simulink model "active_vehicle_ESP_Control"  (R2020a)
settings: Solver=ode4  StartTime=0.0  StopTime=inf  FixedStep=1e-3  RelTol=1e-3
InitFcn:
  | clear mex
model workspace (MAT data in the model file):
  inChnlList : object (value not decoded)
  inChnlListInternal : object (value not decoded)
  outChnlList : object (value not decoded)
  outChnlListInternal : object (value not decoded)
undefined symbols (not defined in the file or in its folder): DiscIntNeverNeededParam, vicrt_initcallback, vicrt_initmexcallback, vicrt_inputfile, vicrt_simulationmanager
libraries: simulink x1
(part 4 of 6)

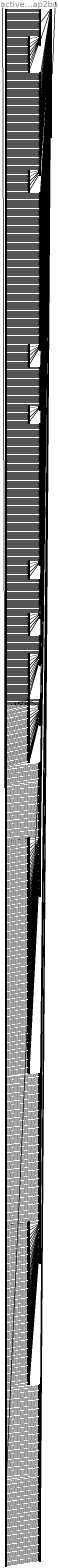
== system active_vehicle_ESP_Control/Vehicle/VI-CarRealTime/Output_Bus/IOmap2bus ==
  In : Inport
  ABS_Activity : BusCreator  Inputs=4
  Actual_Tread_Speed : BusCreator  Inputs=4
  Aggregate_Force_At_Wheel : BusCreator  Inputs=4
  Alpha : BusCreator  Inputs=4
  Animator_Widget : BusCreator  Inputs=2
  Auxiliary_Roll_Force : BusCreator  Inputs=4
  Auxiliary_Roll_Force_at_element : BusCreator  Inputs=2
  Auxiliary_Roll_deformation_at_element : BusCreator  Inputs=2
  Brake : BusCreator  Inputs=8
  Brake_Moment : BusCreator  Inputs=4
  Caster_Angle : BusCreator  Inputs=2
  Chamber_Pressure : BusCreator  Inputs=4
  Contact_Flag : BusCreator  Inputs=4
  Contact_Patch_Global_X : BusCreator  Inputs=4
  Contact_Patch_Global_X1 : BusCreator  Inputs=4
  Contact_Patch_Global_Y : BusCreator  Inputs=4
  Contact_Patch_Global_Y1 : BusCreator  Inputs=4
  Contact_Patch_Global_Z : BusCreator  Inputs=4
  Contact_Patch_Global_Z1 : BusCreator  Inputs=4
  Contact_Patch_Normal_X : BusCreator  Inputs=4
  Contact_Patch_Normal_Y : BusCreator  Inputs=4
  Contact_Patch_Normal_Z : BusCreator  Inputs=4
  Damper : BusCreator  Inputs=5
  Demux : Demux  Outputs=1374
  Drive_Moment : BusCreator  Inputs=4
  Effective_Closing_Speed : BusCreator  Inputs=4
  Effective_Penetration : BusCreator  Inputs=4
  Effective_Rolling_Radius : BusCreator  Inputs=4
  Equivalent_Tread_Speed : BusCreator  Inputs=4
  Euler_Roll : BusCreator  Inputs=4
  External_Friction_Scale_Factor : BusCreator  Inputs=4
  Force_At_Bumper : BusCreator  Inputs=4
  Force_At_Bumper1 : BusCreator  Inputs=4
  Force_At_Damper : BusCreator  Inputs=4
  Force_At_Inerter : BusCreator  Inputs=4
  Force_At_Spring : BusCreator  Inputs=4
  Force_At_Wheel{,1..4} (5 alike) : BusCreator  Inputs=4
  Force_Aux_At_Wheel : BusCreator  Inputs=4
  Global_Omega_X : BusCreator  Inputs=4
  Global_Omega_Y : BusCreator  Inputs=4
  Global_Omega_Z : BusCreator  Inputs=4
  Global_Vx : BusCreator  Inputs=4
  Global_Vy : BusCreator  Inputs=4
  Global_Vz : BusCreator  Inputs=4
  Global_X : BusCreator  Inputs=4
  Global_Y : BusCreator  Inputs=4
  Global_Z : BusCreator  Inputs=4
  Ground_Surface_Contact_Patch_Vx : BusCreator  Inputs=4
  Ground_Surface_Contact_Patch_Vy : BusCreator  Inputs=4
  Ground_Surface_Force_X : BusCreator  Inputs=4
  Ground_Surface_Force_Y : BusCreator  Inputs=4
  Ground_Surface_Force_Z : BusCreator  Inputs=4
  Ground_Surface_Gyroscopic_Moment : BusCreator  Inputs=4
  Ground_Surface_Kappa_Fy : BusCreator  Inputs=4
  Ground_Surface_Moment_X : BusCreator  Inputs=4
  Ground_Surface_Moment_Y : BusCreator  Inputs=4
  Ground_Surface_Moment_Z : BusCreator  Inputs=4
  Ground_Surface_Peak_Friction_X : BusCreator  Inputs=4
  Ground_Surface_Peak_Friction_Y : BusCreator  Inputs=4
  Ground_Surface_Residual_Torque : BusCreator  Inputs=4
  Ground_Surface_Wheel_Center_Vx : BusCreator  Inputs=4
  Gyro : BusCreator  Inputs=10
  Hook_rear : BusCreator  Inputs=18
  Hub_Carrier_Force_Global_X : BusCreator  Inputs=4
  Hub_Carrier_Force_Global_Y : BusCreator  Inputs=4
  Hub_Carrier_Force_Global_Z : BusCreator  Inputs=4
  Hub_Carrier_Force_Local_X : BusCreator  Inputs=4
  Hub_Carrier_Force_Local_Y : BusCreator  Inputs=4
  Hub_Carrier_Force_Local_Z : BusCreator  Inputs=4
  Hub_Carrier_Moment_Global_X : BusCreator  Inputs=4
  Hub_Carrier_Moment_Global_Y : BusCreator  Inputs=4
  Hub_Carrier_Moment_Global_Z : BusCreator  Inputs=4
  Hub_Carrier_Moment_Local_X : BusCreator  Inputs=4
  Hub_Carrier_Moment_Local_Y : BusCreator  Inputs=4
  Hub_Carrier_Moment_Local_Z : BusCreator  Inputs=4
  Hub_Carrier_Omega_X : BusCreator  Inputs=4
  Hub_Carrier_Omega_Y : BusCreator  Inputs=4
  Hub_Carrier_Omega_Z : BusCreator  Inputs=4
  Hub_Carrier_Vx : BusCreator  Inputs=4
  Hub_Carrier_Vy : BusCreator  Inputs=4
  Hub_Carrier_Vz : BusCreator  Inputs=4
  Inclination : BusCreator  Inputs=4
  Inerter : BusCreator  Inputs=5
  Inst_Stiff_Deflection : BusCreator  Inputs=4
  Inst_Stiff_Force : BusCreator  Inputs=4
  Jounce{,1..5} (6 alike) : BusCreator  Inputs=4
  Jounce_Acceleration{,1..3} (4 alike) : BusCreator  Inputs=4
  Jounce_Bumper : BusCreator  Inputs=4
  Jounce_Rate{,1..5} (6 alike) : BusCreator  Inputs=4
  Kingpin_Moment : BusCreator  Inputs=1
  Kingpin_Moment1 : BusCreator  Inputs=2
  Lateral_Relaxation_Length : BusCreator  Inputs=4
  Lateral_Slip_With_Lag : BusCreator  Inputs=4
  Lateral_Slip_Without_Lag : BusCreator  Inputs=4
  Loaded_Radius : BusCreator  Inputs=4
  Locked_Damper_Moment : BusCreator  Inputs=4
  Locked_Moment : BusCreator  Inputs=4
  Locked_Spring_Moment : BusCreator  Inputs=4
  Locked_Switch : BusCreator  Inputs=4
  Lockup_Rotation : BusCreator  Inputs=4
  Longitudinal_Relaxation_Length : BusCreator  Inputs=4
  Longitudinal_Slip_With_Lag : BusCreator  Inputs=4
  Longitudinal_Slip_Without_Lag : BusCreator  Inputs=4
  Moment_Arm_Of_Fx : BusCreator  Inputs=4
  Off_Road_Flag : BusCreator  Inputs=4
  Omega : BusCreator  Inputs=4
  OutputBus : BusCreator  Inputs=113
  PID_CW_At_Spring : BusCreator  Inputs=4
  PID_PH_At_Spring : BusCreator  Inputs=4
  PID_RH_At_Spring : BusCreator  Inputs=4
  Phi : BusCreator  Inputs=4
  Pitch : BusCreator  Inputs=4
  Pneumatic_Trail : BusCreator  Inputs=4
  Pressure : BusCreator  Inputs=4
  Psi : BusCreator  Inputs=4
  Rebound_Bumper : BusCreator  Inputs=4
  Road : BusCreator  Inputs=5
  Road_Material : BusCreator  Inputs=4
  Road_friction : BusCreator  Inputs=4
  Roll : BusCreator  Inputs=2
  Roll_Center_Height : BusCreator  Inputs=2
  Roll_Center_Lateral_Displacement : BusCreator  Inputs=2
  Rotation : BusCreator  Inputs=4
  Sensor : BusCreator  Inputs=16
  Side_View_Angle : BusCreator  Inputs=4
  Spindle_Steer : BusCreator  Inputs=4
  Spring : BusCreator  Inputs=10
  Steering_Instant_Axis_Rotation : BusCreator  Inputs=2
  Steering_System : BusCreator  Inputs=7
  Suspension : BusCreator  Inputs=16
  System : BusCreator  Inputs=17
  System_Mass_Center : BusCreator  Inputs=13
  Temperature_1 : BusCreator  Inputs=4
  Temperature_2 : BusCreator  Inputs=4
  Temperature_3 : BusCreator  Inputs=4
  Theta : BusCreator  Inputs=4
  TieRod_Force_Left : BusCreator  Inputs=3
  TieRod_Force_Right : BusCreator  Inputs=3
  Tire : BusCreator  Inputs=52
  User_Input_Contact_Patch_Global_Z_Perturbation : BusCreator  Inputs=4
  Vehicle : BusCreator  Inputs=46
  Vehicle_States : BusCreator  Inputs=20
  Wheel : BusCreator  Inputs=37
  Yaw : BusCreator  Inputs=4
  aero_forces : BusCreator  Inputs=24
  base_acceleration : BusCreator  Inputs=4
  base_deformation : BusCreator  Inputs=4
  base_velocity : BusCreator  Inputs=4
  bul_jounce_stop_data : BusCreator  Inputs=6
  bul_rebound_stop_data : BusCreator  Inputs=6
  bur_jounce_stop_data : BusCreator  Inputs=6
  bur_rebound_stop_data : BusCreator  Inputs=6
  bus_dmp_jounce_stop_data : BusCreator  Inputs=6
  bus_ins_jounce_stop_data : BusCreator  Inputs=6
  bus_roll_dmp_jounce_stop_data : BusCreator  Inputs=6
  bus_spr_jounce_stop_data : BusCreator  Inputs=6
  chassis_accelerations : BusCreator  Inputs=6
  chassis_displacements : BusCreator  Inputs=9
  chassis_velocities : BusCreator  Inputs=6
  clutch : BusCreator  Inputs=8
  condition_sensors : BusCreator  Inputs=1
  cp_force_lateralFL : BusCreator  Inputs=3
  cp_force_lateralFR : BusCreator  Inputs=3
  cp_force_lateralRL : BusCreator  Inputs=3
  cp_force_lateralRR : BusCreator  Inputs=3
  cp_force_longitudinalFL : BusCreator  Inputs=3
  cp_force_longitudinalFR : BusCreator  Inputs=3
  cp_force_longitudinalRL : BusCreator  Inputs=3
  cp_force_longitudinalRR : BusCreator  Inputs=3
  cp_force_normalFL : BusCreator  Inputs=3
  cp_force_normalFR : BusCreator  Inputs=3
  cp_force_normalRL : BusCreator  Inputs=3
  cp_force_normalRR : BusCreator  Inputs=3
  cross_weight : BusCreator  Inputs=4
  dal_ride_damper_data : BusCreator  Inputs=4
  dar_ride_damper_data : BusCreator  Inputs=4
  das_ride_damper_data : BusCreator  Inputs=6
  das_roll_damper_data : BusCreator  Inputs=8
  das_third_damper_data : BusCreator  Inputs=6
  differential_central : BusCreator  Inputs=7
  differential_front : BusCreator  Inputs=7
  differential_rear : BusCreator  Inputs=7
  differential_speeds : BusCreator  Inputs=9
  differential_torques : BusCreator  Inputs=9
  driver_demands : BusCreator  Inputs=7
  driving_machine_monitor : BusCreator  Inputs=15
  engine : BusCreator  Inputs=11
  fuel_consumption : BusCreator  Inputs=4
  ges_chassis_XFORM : BusCreator  Inputs=6
  ges_hub_XFORMFL : BusCreator  Inputs=6
  ges_hub_XFORMFR : BusCreator  Inputs=6
  ges_hub_XFORMRL : BusCreator  Inputs=6
  ges_hub_XFORMRR : BusCreator  Inputs=6
  hub2cp_XFORMFL : BusCreator  Inputs=3
  hub2cp_XFORMFR : BusCreator  Inputs=3
  hub2cp_XFORMRL : BusCreator  Inputs=3
  hub2cp_XFORMRR : BusCreator  Inputs=3
  hub_center_accx : BusCreator  Inputs=4
  hub_center_accy : BusCreator  Inputs=4
  hub_center_accz : BusCreator  Inputs=4
  inl_ride_inerter_data : BusCreator  Inputs=6
  inr_ride_inerter_data : BusCreator  Inputs=6
  ins_inerter_data : BusCreator  Inputs=10
  jfs_torsional_stiffness_data : BusCreator  Inputs=12
  motor_to_central_differential : BusCreator  Inputs=11
  motor_to_clutch : BusCreator  Inputs=11
  motor_to_front_differential : BusCreator  Inputs=11
  motor_to_front_left_wheel : BusCreator  Inputs=11
  motor_to_front_right_wheel : BusCreator  Inputs=11
  motor_to_gearbox : BusCreator  Inputs=11
  motor_to_rear_differential : BusCreator  Inputs=11
  motor_to_rear_left_wheel : BusCreator  Inputs=11
  motor_to_rear_right_wheel : BusCreator  Inputs=11
  nsl_ride_spring_data : BusCreator  Inputs=6
  nsr_ride_spring_data : BusCreator  Inputs=6
  nss_ride_spring_data : BusCreator  Inputs=10
  res_dmp_rebound_stop_data : BusCreator  Inputs=6
  res_ins_rebound_stop_data : BusCreator  Inputs=6
  res_roll_dmp_rebound_stop_data : BusCreator  Inputs=6
  res_spr_rebound_stop_data : BusCreator  Inputs=6
  rhl_front_setup_sensor_data : BusCreator  Inputs=1
  rhl_rear_setup_sensor_data : BusCreator  Inputs=1
  rhr_front_setup_sensor_data : BusCreator  Inputs=1
  rhr_rear_setup_sensor_data : BusCreator  Inputs=1
  rhs_front_setup_sensor_data : BusCreator  Inputs=1
  rhs_rear_setup_sensor_data : BusCreator  Inputs=1
  til_wheel_tire_forces : BusCreator  Inputs=18
  til_wheel_tire_kinematics : BusCreator  Inputs=9
  til_wheel_tire_rolling_states : BusCreator  Inputs=9
  tir_wheel_tire_forces : BusCreator  Inputs=18
  tir_wheel_tire_kinematics : BusCreator  Inputs=9
  tir_wheel_tire_rolling_states : BusCreator  Inputs=9
  torque_converter : BusCreator  Inputs=9
  transmission : BusCreator  Inputs=10
  ues_third_spring_data : BusCreator  Inputs=6
  upright_accelerometer : BusCreator  Inputs=4
  wheel_angles : BusCreator  Inputs=24
  wheel_center_dispx : BusCreator  Inputs=4
  wheel_center_dispy : BusCreator  Inputs=4
  wheel_center_dispz : BusCreator  Inputs=4
  whl_front_wheel_XFORM : BusCreator  Inputs=9
  whl_rear_wheel_XFORM : BusCreator  Inputs=9
  whl_twin_rear_wheel_XFORM : BusCreator  Inputs=9
  whr_front_wheel_XFORM : BusCreator  Inputs=9
  whr_rear_wheel_XFORM : BusCreator  Inputs=9
  whr_twin_rear_wheel_XFORM : BusCreator  Inputs=9
  Out : Outport
  wires:
  In/1 -> Demux/1
  OutputBus/1 -> Out/1  "OutputBus"
  aero_forces/1 -> OutputBus/1  "aero_forces"
  Demux/1 -> aero_forces/1  "aero_balance"
  Demux/2 -> aero_forces/2  "center_downforce"
  Demux/3 -> aero_forces/3  "center_sideforce"
  Demux/4 -> aero_forces/4  "drag_arm"
  Demux/5 -> aero_forces/5  "drag_force"
  Demux/6 -> aero_forces/6  "drag_force_front"
  Demux/7 -> aero_forces/7  "drag_force_rear"
  Demux/8 -> aero_forces/8  "drag_torque"
  Demux/9 -> aero_forces/9  "front_downforce"
  Demux/10 -> aero_forces/10  "front_sideforce"
  Demux/11 -> aero_forces/11  "height_auxiliary"
  Demux/12 -> aero_forces/12  "height_front"
  Demux/13 -> aero_forces/13  "height_rear"
  Demux/14 -> aero_forces/14  "lateral_velocity"
  Demux/15 -> aero_forces/15  "longitudinal_velocity"
  Demux/16 -> aero_forces/16  "pitch"
  Demux/17 -> aero_forces/17  "rear_downforce"
  Demux/18 -> aero_forces/18  "rear_sideforce"
  Demux/19 -> aero_forces/19  "roll"
  Demux/20 -> aero_forces/20  "roll_torque"
  Demux/21 -> aero_forces/21  "side_slip"
  Demux/22 -> aero_forces/22  "steer"
  Demux/23 -> aero_forces/23  "vertical_velocity"
  Demux/24 -> aero_forces/24  "yaw_torque"
  Brake/1 -> OutputBus/2  "Brake"
  ABS_Activity/1 -> Brake/1  "ABS_Activity"
  Demux/25 -> ABS_Activity/1  "L1"
  Demux/26 -> ABS_Activity/2  "L2"
  Demux/27 -> ABS_Activity/3  "R1"
  Demux/28 -> ABS_Activity/4  "R2"
  Brake_Moment/1 -> Brake/2  "Brake_Moment"
  Demux/29 -> Brake_Moment/1  "L1"
  Demux/30 -> Brake_Moment/2  "L2"
  Demux/31 -> Brake_Moment/3  "R1"
  Demux/32 -> Brake_Moment/4  "R2"
  Chamber_Pressure/1 -> Brake/3  "Chamber_Pressure"
  Demux/33 -> Chamber_Pressure/1  "L1"
  Demux/34 -> Chamber_Pressure/2  "L2"
  Demux/35 -> Chamber_Pressure/3  "R1"
  Demux/36 -> Chamber_Pressure/4  "R2"
  Locked_Damper_Moment/1 -> Brake/4  "Locked_Damper_Moment"
  Demux/37 -> Locked_Damper_Moment/1  "L1"
  Demux/38 -> Locked_Damper_Moment/2  "L2"
  Demux/39 -> Locked_Damper_Moment/3  "R1"
  Demux/40 -> Locked_Damper_Moment/4  "R2"
  Locked_Moment/1 -> Brake/5  "Locked_Moment"
  Demux/41 -> Locked_Moment/1  "L1"
  Demux/42 -> Locked_Moment/2  "L2"
  Demux/43 -> Locked_Moment/3  "R1"
  Demux/44 -> Locked_Moment/4  "R2"
  Locked_Spring_Moment/1 -> Brake/6  "Locked_Spring_Moment"
  Demux/45 -> Locked_Spring_Moment/1  "L1"
  Demux/46 -> Locked_Spring_Moment/2  "L2"
  Demux/47 -> Locked_Spring_Moment/3  "R1"
  Demux/48 -> Locked_Spring_Moment/4  "R2"
  Locked_Switch/1 -> Brake/7  "Locked_Switch"
  Demux/49 -> Locked_Switch/1  "L1"
  Demux/50 -> Locked_Switch/2  "L2"
  Demux/51 -> Locked_Switch/3  "R1"
  Demux/52 -> Locked_Switch/4  "R2"
  Lockup_Rotation/1 -> Brake/8  "Lockup_Rotation"
  Demux/53 -> Lockup_Rotation/1  "L1"
  Demux/54 -> Lockup_Rotation/2  "L2"
  Demux/55 -> Lockup_Rotation/3  "R1"
  Demux/56 -> Lockup_Rotation/4  "R2"
  bul_jounce_stop_data/1 -> OutputBus/3  "bul_jounce_stop_data"
  Demux/57 -> bul_jounce_stop_data/1  "force_front"
  Demux/58 -> bul_jounce_stop_data/2  "force_rear"
  Demux/59 -> bul_jounce_stop_data/3  "jounce_front"
  Demux/60 -> bul_jounce_stop_data/4  "jounce_rear"
  Demux/61 -> bul_jounce_stop_data/5  "velocity_front"
  Demux/62 -> bul_jounce_stop_data/6  "velocity_rear"
  bul_rebound_stop_data/1 -> OutputBus/4  "bul_rebound_stop_data"
  Demux/63 -> bul_rebound_stop_data/1  "force_front"
  Demux/64 -> bul_rebound_stop_data/2  "force_rear"
  Demux/65 -> bul_rebound_stop_data/3  "jounce_front"
  Demux/66 -> bul_rebound_stop_data/4  "jounce_rear"
  Demux/67 -> bul_rebound_stop_data/5  "velocity_front"
  Demux/68 -> bul_rebound_stop_data/6  "velocity_rear"
  bur_jounce_stop_data/1 -> OutputBus/5  "bur_jounce_stop_data"
  Demux/69 -> bur_jounce_stop_data/1  "force_front"
  Demux/70 -> bur_jounce_stop_data/2  "force_rear"
  Demux/71 -> bur_jounce_stop_data/3  "jounce_front"
  Demux/72 -> bur_jounce_stop_data/4  "jounce_rear"
  Demux/73 -> bur_jounce_stop_data/5  "velocity_front"
  Demux/74 -> bur_jounce_stop_data/6  "velocity_rear"
  bur_rebound_stop_data/1 -> OutputBus/6  "bur_rebound_stop_data"
  Demux/75 -> bur_rebound_stop_data/1  "force_front"
  Demux/76 -> bur_rebound_stop_data/2  "force_rear"
  Demux/77 -> bur_rebound_stop_data/3  "jounce_front"
  Demux/78 -> bur_rebound_stop_data/4  "jounce_rear"
  Demux/79 -> bur_rebound_stop_data/5  "velocity_front"
  Demux/80 -> bur_rebound_stop_data/6  "velocity_rear"
  bus_dmp_jounce_stop_data/1 -> OutputBus/7  "bus_dmp_jounce_stop_data"
  Demux/81 -> bus_dmp_jounce_stop_data/1  "displacement_front"
  Demux/82 -> bus_dmp_jounce_stop_data/2  "displacement_rear"
  Demux/83 -> bus_dmp_jounce_stop_data/3  "force_front"
  Demux/84 -> bus_dmp_jounce_stop_data/4  "force_rear"
  Demux/85 -> bus_dmp_jounce_stop_data/5  "velocity_front"
  Demux/86 -> bus_dmp_jounce_stop_data/6  "velocity_rear"
  bus_ins_jounce_stop_data/1 -> OutputBus/8  "bus_ins_jounce_stop_data"
  Demux/87 -> bus_ins_jounce_stop_data/1  "displacement_front"
  Demux/88 -> bus_ins_jounce_stop_data/2  "displacement_rear"
  Demux/89 -> bus_ins_jounce_stop_data/3  "force_front"
  Demux/90 -> bus_ins_jounce_stop_data/4  "force_rear"
  Demux/91 -> bus_ins_jounce_stop_data/5  "velocity_front"
  Demux/92 -> bus_ins_jounce_stop_data/6  "velocity_rear"
  bus_roll_dmp_jounce_stop_data/1 -> OutputBus/9  "bus_roll_dmp_jounce_stop_data"
  Demux/93 -> bus_roll_dmp_jounce_stop_data/1  "displacement_front"
  Demux/94 -> bus_roll_dmp_jounce_stop_data/2  "displacement_rear"
  Demux/95 -> bus_roll_dmp_jounce_stop_data/3  "force_front"
  Demux/96 -> bus_roll_dmp_jounce_stop_data/4  "force_rear"
  Demux/97 -> bus_roll_dmp_jounce_stop_data/5  "velocity_front"
  Demux/98 -> bus_roll_dmp_jounce_stop_data/6  "velocity_rear"
  bus_spr_jounce_stop_data/1 -> OutputBus/10  "bus_spr_jounce_stop_data"
  Demux/99 -> bus_spr_jounce_stop_data/1  "displacement_front"
  Demux/100 -> bus_spr_jounce_stop_data/2  "displacement_rear"
  Demux/101 -> bus_spr_jounce_stop_data/3  "force_front"
  Demux/102 -> bus_spr_jounce_stop_data/4  "force_rear"
  Demux/103 -> bus_spr_jounce_stop_data/5  "velocity_front"
  Demux/104 -> bus_spr_jounce_stop_data/6  "velocity_rear"
  chassis_accelerations/1 -> OutputBus/11  "chassis_accelerations"
  Demux/105 -> chassis_accelerations/1  "lateral"
  Demux/106 -> chassis_accelerations/2  "longitudinal"
  Demux/107 -> chassis_accelerations/3  "pitch"
  Demux/108 -> chassis_accelerations/4  "roll"
  Demux/109 -> chassis_accelerations/5  "vertical"
  Demux/110 -> chassis_accelerations/6  "yaw"
  chassis_displacements/1 -> OutputBus/12  "chassis_displacements"
  Demux/111 -> chassis_displacements/1  "lateral"
  Demux/112 -> chassis_displacements/2  "longitudinal"
  Demux/113 -> chassis_displacements/3  "pitch"
  Demux/114 -> chassis_displacements/4  "pitch_wrt_road"
  Demux/115 -> chassis_displacements/5  "roll"
  Demux/116 -> chassis_displacements/6  "roll_wrt_road"
  Demux/117 -> chassis_displacements/7  "vertical"
  Demux/118 -> chassis_displacements/8  "vertical_wrt_road"
  Demux/119 -> chassis_displacements/9  "yaw"
  chassis_velocities/1 -> OutputBus/13  "chassis_velocities"
  Demux/120 -> chassis_velocities/1  "lateral"
  Demux/121 -> chassis_velocities/2  "longitudinal"
  Demux/122 -> chassis_velocities/3  "pitch"
  Demux/123 -> chassis_velocities/4  "roll"
  Demux/124 -> chassis_velocities/5  "vertical"
  Demux/125 -> chassis_velocities/6  "yaw"
  clutch/1 -> OutputBus/14  "clutch"
  Demux/126 -> clutch/1  "clutch_rpm"
  Demux/127 -> clutch/2  "effective_clutch"
  Demux/128 -> clutch/3  "gearbox_inputshaft_alpha"
  Demux/129 -> clutch/4  "gearbox_inputshaft_angle"
  Demux/130 -> clutch/5  "gearbox_inputshaft_omega"
  Demux/131 -> clutch/6  "inputplate_torque"
  Demux/132 -> clutch/7  "slip_angle"
  Demux/133 -> clutch/8  "torque"
  condition_sensors/1 -> OutputBus/15  "condition_sensors"
  Demux/134 -> condition_sensors/1  "side_slip_angle"
  cross_weight/1 -> OutputBus/16  "cross_weight"
  Demux/135 -> cross_weight/1  "crossL1R2_ratio"
  Demux/136 -> cross_weight/2  "crossR1L2_ratio"
  Demux/137 -> cross_weight/3  "nose_ratio"
  Demux/138 -> cross_weight/4  "side_right_ratio"
  dal_ride_damper_data/1 -> OutputBus/17  "dal_ride_damper_data"
  Demux/139 -> dal_ride_damper_data/1  "force_front"
  Demux/140 -> dal_ride_damper_data/2  "force_rear"
  Demux/141 -> dal_ride_damper_data/3  "velocity_front"
  Demux/142 -> dal_ride_damper_data/4  "velocity_rear"
  Damper/1 -> OutputBus/18  "Damper"
  Force_At_Damper/1 -> Damper/1  "Force_At_Damper"
  Demux/143 -> Force_At_Damper/1  "L1"
  Demux/144 -> Force_At_Damper/2  "L2"
  Demux/145 -> Force_At_Damper/3  "R1"
  Demux/146 -> Force_At_Damper/4  "R2"
  Force_At_Wheel/1 -> Damper/2  "Force_At_Wheel"
  Demux/147 -> Force_At_Wheel/1  "L1"
  Demux/148 -> Force_At_Wheel/2  "L2"
  Demux/149 -> Force_At_Wheel/3  "R1"
  Demux/150 -> Force_At_Wheel/4  "R2"
  Jounce/1 -> Damper/3  "Jounce"
  Demux/151 -> Jounce/1  "L1"
  Demux/152 -> Jounce/2  "L2"
  Demux/153 -> Jounce/3  "R1"
  Demux/154 -> Jounce/4  "R2"
  Jounce_Acceleration/1 -> Damper/4  "Jounce_Acceleration"
  Demux/155 -> Jounce_Acceleration/1  "L1"
  Demux/156 -> Jounce_Acceleration/2  "L2"
  Demux/157 -> Jounce_Acceleration/3  "R1"
  Demux/158 -> Jounce_Acceleration/4  "R2"
  Jounce_Rate/1 -> Damper/5  "Jounce_Rate"
  Demux/159 -> Jounce_Rate/1  "L1"
  Demux/160 -> Jounce_Rate/2  "L2"
  Demux/161 -> Jounce_Rate/3  "R1"
  Demux/162 -> Jounce_Rate/4  "R2"
  dar_ride_damper_data/1 -> OutputBus/19  "dar_ride_damper_data"
  Demux/163 -> dar_ride_damper_data/1  "force_front"
  Demux/164 -> dar_ride_damper_data/2  "force_rear"
  Demux/165 -> dar_ride_damper_data/3  "velocity_front"
  Demux/166 -> dar_ride_damper_data/4  "velocity_rear"
  das_ride_damper_data/1 -> OutputBus/20  "das_ride_damper_data"
  Demux/167 -> das_ride_damper_data/1  "displacement_front"
  Demux/168 -> das_ride_damper_data/2  "displacement_rear"
  Demux/169 -> das_ride_damper_data/3  "force_front"
  Demux/170 -> das_ride_damper_data/4  "force_rear"
  Demux/171 -> das_ride_damper_data/5  "velocity_front"
  Demux/172 -> das_ride_damper_data/6  "velocity_rear"
  das_roll_damper_data/1 -> OutputBus/21  "das_roll_damper_data"
  Demux/173 -> das_roll_damper_data/1  "displacement_front"
  Demux/174 -> das_roll_damper_data/2  "displacement_rear"
  Demux/175 -> das_roll_damper_data/3  "force_at_wheel_front"
  Demux/176 -> das_roll_damper_data/4  "force_at_wheel_rear"
  Demux/177 -> das_roll_damper_data/5  "force_front"
  Demux/178 -> das_roll_damper_data/6  "force_rear"
  Demux/179 -> das_roll_damper_data/7  "velocity_front"
  Demux/180 -> das_roll_damper_data/8  "velocity_rear"
  das_third_damper_data/1 -> OutputBus/22  "das_third_damper_data"
  Demux/181 -> das_third_damper_data/1  "displacement_front"
  Demux/182 -> das_third_damper_data/2  "displacement_rear"
  Demux/183 -> das_third_damper_data/3  "force_front"
  Demux/184 -> das_third_damper_data/4  "force_rear"
  Demux/185 -> das_third_damper_data/5  "velocity_front"
  Demux/186 -> das_third_damper_data/6  "velocity_rear"
  differential_central/1 -> OutputBus/23  "differential_central"
  Demux/187 -> differential_central/1  "diff_front_inputshaft_alpha"
  Demux/188 -> differential_central/2  "diff_front_inputshaft_angle"
  Demux/189 -> differential_central/3  "diff_front_inputshaft_omega"
  Demux/190 -> differential_central/4  "diff_rear_inputshaft_alpha"
  Demux/191 -> differential_central/5  "diff_rear_inputshaft_angle"
  Demux/192 -> differential_central/6  "diff_rear_inputshaft_omega"
  Demux/193 -> differential_central/7  "gearbox_outputshaft_torque"
  differential_front/1 -> OutputBus/24  "differential_front"
  Demux/194 -> differential_front/1  "diff_central_front_outputshaft_torque"
  Demux/195 -> differential_front/2  "wheel_front_left_alpha"
  Demux/196 -> differential_front/3  "wheel_front_left_angle"
  Demux/197 -> differential_front/4  "wheel_front_left_omega"
  Demux/198 -> differential_front/5  "wheel_front_right_alpha"
  Demux/199 -> differential_front/6  "wheel_front_right_angle"
  Demux/200 -> differential_front/7  "wheel_front_right_omega"
  differential_rear/1 -> OutputBus/25  "differential_rear"
  Demux/201 -> differential_rear/1  "diff_central_rear_outputshaft_torque"
  Demux/202 -> differential_rear/2  "wheel_rear_left_alpha"
  Demux/203 -> differential_rear/3  "wheel_rear_left_angle"
  Demux/204 -> differential_rear/4  "wheel_rear_left_omega"
  Demux/205 -> differential_rear/5  "wheel_rear_right_alpha"
  Demux/206 -> differential_rear/6  "wheel_rear_right_angle"
  Demux/207 -> differential_rear/7  "wheel_rear_right_omega"
  differential_speeds/1 -> OutputBus/26  "differential_speeds"
  Demux/208 -> differential_speeds/1  "halfshaft_omega_central_front"
  Demux/209 -> differential_speeds/2  "halfshaft_omega_central_rear"
  Demux/210 -> differential_speeds/3  "halfshaft_omega_delta_central"
  Demux/211 -> differential_speeds/4  "halfshaft_omega_delta_front"
  Demux/212 -> differential_speeds/5  "halfshaft_omega_delta_rear"
  Demux/213 -> differential_speeds/6  "halfshaft_omega_left_front"
  Demux/214 -> differential_speeds/7  "halfshaft_omega_left_rear"
  Demux/215 -> differential_speeds/8  "halfshaft_omega_right_front"
  Demux/216 -> differential_speeds/9  "halfshaft_omega_right_rear"
  differential_torques/1 -> OutputBus/27  "differential_torques"
  Demux/217 -> differential_torques/1  "differential_torque_central"
  Demux/218 -> differential_torques/2  "differential_torque_front"
  Demux/219 -> differential_torques/3  "differential_torque_rear"
  Demux/220 -> differential_torques/4  "output_torque_central_front"
  Demux/221 -> differential_torques/5  "output_torque_central_rear"
  Demux/222 -> differential_torques/6  "output_torque_left_front"
  Demux/223 -> differential_torques/7  "output_torque_left_rear"
  Demux/224 -> differential_torques/8  "output_torque_right_front"
  Demux/225 -> differential_torques/9  "output_torque_right_rear"
  driver_demands/1 -> OutputBus/28  "driver_demands"
  Demux/226 -> driver_demands/1  "brake"
  Demux/227 -> driver_demands/2  "brake_pressure"
  Demux/228 -> driver_demands/3  "clutch"
  Demux/229 -> driver_demands/4  "gear"
  Demux/230 -> driver_demands/5  "steering"
  Demux/231 -> driver_demands/6  "steering_velocity"
  Demux/232 -> driver_demands/7  "throttle"
  driving_machine_monitor/1 -> OutputBus/29  "driving_machine_monitor"
  Demux/233 -> driving_machine_monitor/1  "driver_brake"
  Demux/234 -> driving_machine_monitor/2  "driver_clutch"
  Demux/235 -> driving_machine_monitor/3  "driver_gear"
  Demux/236 -> driving_machine_monitor/4  "driver_steering"
  Demux/237 -> driving_machine_monitor/5  "driver_throttle"
  Demux/238 -> driving_machine_monitor/6  "maneuver_ID"
  Demux/239 -> driving_machine_monitor/7  "path_curvature"
  Demux/240 -> driving_machine_monitor/8  "path_distance"
  Demux/241 -> driving_machine_monitor/9  "path_s"
  Demux/242 -> driving_machine_monitor/10  "path_x"
  Demux/243 -> driving_machine_monitor/11  "path_y"
  Demux/244 -> driving_machine_monitor/12  "path_z"
  Demux/245 -> driving_machine_monitor/13  "target_ax"
  Demux/246 -> driving_machine_monitor/14  "target_engine_torque"
  Demux/247 -> driving_machine_monitor/15  "target_vx"
  engine/1 -> OutputBus/30  "engine"
  Demux/248 -> engine/1  "clutch_inputplate_alpha"
  Demux/249 -> engine/2  "clutch_inputplate_angle"
  Demux/250 -> engine/3  "clutch_inputplate_omega"
  Demux/251 -> engine/4  "effective_throttle"
  Demux/252 -> engine/5  "engine_rpm"
  Demux/253 -> engine/6  "Max_Engine_torque"
  Demux/254 -> engine/7  "Min_engine_torque"
  Demux/255 -> engine/8  "Power_HP"
  Demux/256 -> engine/9  "Power_KW"
  Demux/257 -> engine/10  "TCS_activity"
  Demux/258 -> engine/11  "torque"
  fuel_consumption/1 -> OutputBus/31  "fuel_consumption"
  Demux/259 -> fuel_consumption/1  "BSFC"
  Demux/260 -> fuel_consumption/2  "instantaneous"
  Demux/261 -> fuel_consumption/3  "instantaneous_Liter_100km"
  Demux/262 -> fuel_consumption/4  "overall"
  ges_chassis_XFORM/1 -> OutputBus/32  "ges_chassis_XFORM"
  Demux/263 -> ges_chassis_XFORM/1  "Phi"
  Demux/264 -> ges_chassis_XFORM/2  "Psi"
  Demux/265 -> ges_chassis_XFORM/3  "Theta"
  Demux/266 -> ges_chassis_XFORM/4  "X"
  Demux/267 -> ges_chassis_XFORM/5  "Y"
  Demux/268 -> ges_chassis_XFORM/6  "Z"
  Gyro/1 -> OutputBus/33  "Gyro"
  Demux/269 -> Gyro/1  "Driver_X"
  Demux/270 -> Gyro/2  "Driver_Z"
  Demux/271 -> Gyro/3  "gyro_ACCX"
  Demux/272 -> Gyro/4  "gyro_ACCY"
  Demux/273 -> Gyro/5  "gyro_VX"
  Demux/274 -> Gyro/6  "gyro_X"
  Demux/275 -> Gyro/7  "gyro_Y"
  Demux/276 -> Gyro/8  "sensor_1_Z"
  Demux/277 -> Gyro/9  "sensor_2_Z"
  Demux/278 -> Gyro/10  "sensor_3_Z"
  Hook_rear/1 -> OutputBus/34  "Hook_rear"
  Demux/279 -> Hook_rear/1  "Global_force_X"
  Demux/280 -> Hook_rear/2  "Global_force_Y"
  Demux/281 -> Hook_rear/3  "Global_force_Z"
  Demux/282 -> Hook_rear/4  "Global_Moment_X"
  Demux/283 -> Hook_rear/5  "Global_Moment_Y"
  Demux/284 -> Hook_rear/6  "Global_Moment_Z"
  Demux/285 -> Hook_rear/7  "Hook_Phi"
  Demux/286 -> Hook_rear/8  "Hook_Psi"
  Demux/287 -> Hook_rear/9  "Hook_Theta"
  Demux/288 -> Hook_rear/10  "Hook_X"
  Demux/289 -> Hook_rear/11  "Hook_Y"
  Demux/290 -> Hook_rear/12  "Hook_Z"
  Demux/291 -> Hook_rear/13  "Local_force_X"
  Demux/292 -> Hook_rear/14  "Local_force_Y"
  Demux/293 -> Hook_rear/15  "Local_force_Z"
  Demux/294 -> Hook_rear/16  "Local_Moment_X"
  Demux/295 -> Hook_rear/17  "Local_Moment_Y"
  Demux/296 -> Hook_rear/18  "Local_Moment_Z"
  Inerter/1 -> OutputBus/35  "Inerter"
  Force_At_Inerter/1 -> Inerter/1  "Force_At_Inerter"
  Demux/297 -> Force_At_Inerter/1  "L1"
  Demux/298 -> Force_At_Inerter/2  "L2"
  Demux/299 -> Force_At_Inerter/3  "R1"
  Demux/300 -> Force_At_Inerter/4  "R2"
  Force_At_Wheel1/1 -> Inerter/2  "Force_At_Wheel"
  Demux/301 -> Force_At_Wheel1/1  "L1"
  Demux/302 -> Force_At_Wheel1/2  "L2"
  Demux/303 -> Force_At_Wheel1/3  "R1"
  Demux/304 -> Force_At_Wheel1/4  "R2"
  Jounce1/1 -> Inerter/3  "Jounce"
  Demux/305 -> Jounce1/1  "L1"
  Demux/306 -> Jounce1/2  "L2"
  Demux/307 -> Jounce1/3  "R1"
  Demux/308 -> Jounce1/4  "R2"
  Jounce_Acceleration1/1 -> Inerter/4  "Jounce_Acceleration"
  Demux/309 -> Jounce_Acceleration1/1  "L1"
  Demux/310 -> Jounce_Acceleration1/2  "L2"
  Demux/311 -> Jounce_Acceleration1/3  "R1"
  Demux/312 -> Jounce_Acceleration1/4  "R2"
  Jounce_Rate1/1 -> Inerter/5  "Jounce_Rate"
  Demux/313 -> Jounce_Rate1/1  "L1"
  Demux/314 -> Jounce_Rate1/2  "L2"
  Demux/315 -> Jounce_Rate1/3  "R1"
  Demux/316 -> Jounce_Rate1/4  "R2"
  inl_ride_inerter_data/1 -> OutputBus/36  "inl_ride_inerter_data"
  Demux/317 -> inl_ride_inerter_data/1  "acceleration_front"
  Demux/318 -> inl_ride_inerter_data/2  "acceleration_rear"
  Demux/319 -> inl_ride_inerter_data/3  "displacement_front"
  Demux/320 -> inl_ride_inerter_data/4  "displacement_rear"
  Demux/321 -> inl_ride_inerter_data/5  "force_front"
  Demux/322 -> inl_ride_inerter_data/6  "force_rear"
  inr_ride_inerter_data/1 -> OutputBus/37  "inr_ride_inerter_data"
  Demux/323 -> inr_ride_inerter_data/1  "acceleration_front"
  Demux/324 -> inr_ride_inerter_data/2  "acceleration_rear"
  Demux/325 -> inr_ride_inerter_data/3  "displacement_front"
  Demux/326 -> inr_ride_inerter_data/4  "displacement_rear"
  Demux/327 -> inr_ride_inerter_data/5  "force_front"
  Demux/328 -> inr_ride_inerter_data/6  "force_rear"
  ins_inerter_data/1 -> OutputBus/38  "ins_inerter_data"
  Demux/329 -> ins_inerter_data/1  "acceleration_front"
  Demux/330 -> ins_inerter_data/2  "acceleration_rear"
  Demux/331 -> ins_inerter_data/3  "displacement_front"
  Demux/332 -> ins_inerter_data/4  "displacement_rear"
  Demux/333 -> ins_inerter_data/5  "force_at_wheel_front"
  Demux/334 -> ins_inerter_data/6  "force_at_wheel_rear"
  Demux/335 -> ins_inerter_data/7  "force_front"
  Demux/336 -> ins_inerter_data/8  "force_rear"
  Demux/337 -> ins_inerter_data/9  "velocity_front"
  Demux/338 -> ins_inerter_data/10  "velocity_rear"
  jfs_torsional_stiffness_data/1 -> OutputBus/39  "jfs_torsional_stiffness_data"
  Demux/339 -> jfs_torsional_stiffness_data/1  "AX_1"
  Demux/340 -> jfs_torsional_stiffness_data/2  "AY_1"
  Demux/341 -> jfs_torsional_stiffness_data/3  "AZ_1"
  Demux/342 -> jfs_torsional_stiffness_data/4  "FX_1"
  Demux/343 -> jfs_torsional_stiffness_data/5  "FY_1"
  Demux/344 -> jfs_torsional_stiffness_data/6  "FZ_1"
  Demux/345 -> jfs_torsional_stiffness_data/7  "TX_1"
  Demux/346 -> jfs_torsional_stiffness_data/8  "TY_1"
  Demux/347 -> jfs_torsional_stiffness_data/9  "TZ_1"
  Demux/348 -> jfs_torsional_stiffness_data/10  "X_1"
  Demux/349 -> jfs_torsional_stiffness_data/11  "Y_1"
  Demux/350 -> jfs_torsional_stiffness_data/12  "Z_1"
  Jounce_Bumper/1 -> OutputBus/40  "Jounce_Bumper"
  Force_At_Bumper/1 -> Jounce_Bumper/1  "Force_At_Bumper"
  Demux/351 -> Force_At_Bumper/1  "L1"
  Demux/352 -> Force_At_Bumper/2  "L2"
  Demux/353 -> Force_At_Bumper/3  "R1"
  Demux/354 -> Force_At_Bumper/4  "R2"
  Force_At_Wheel2/1 -> Jounce_Bumper/2  "Force_At_Wheel"
  Demux/355 -> Force_At_Wheel2/1  "L1"
  Demux/356 -> Force_At_Wheel2/2  "L2"
  Demux/357 -> Force_At_Wheel2/3  "R1"
  Demux/358 -> Force_At_Wheel2/4  "R2"
  Jounce2/1 -> Jounce_Bumper/3  "Jounce"
  Demux/359 -> Jounce2/1  "L1"
  Demux/360 -> Jounce2/2  "L2"
  Demux/361 -> Jounce2/3  "R1"
  Demux/362 -> Jounce2/4  "R2"
  Jounce_Rate2/1 -> Jounce_Bumper/4  "Jounce_Rate"
  Demux/363 -> Jounce_Rate2/1  "L1"
  Demux/364 -> Jounce_Rate2/2  "L2"
  Demux/365 -> Jounce_Rate2/3  "R1"
  Demux/366 -> Jounce_Rate2/4  "R2"
  motor_to_central_differential/1 -> OutputBus/41  "motor_to_central_differential"
  Demux/367 -> motor_to_central_differential/1  "differential_inputshaft_alpha"
  Demux/368 -> motor_to_central_differential/2  "differential_inputshaft_angle"
  Demux/369 -> motor_to_central_differential/3  "differential_inputshaft_omega"
  Demux/370 -> motor_to_central_differential/4  "effective_throttle"
  Demux/371 -> motor_to_central_differential/5  "engine_rpm"
  Demux/372 -> motor_to_central_differential/6  "Max_Engine_torque"
  Demux/373 -> motor_to_central_differential/7  "Min_engine_torque"
  Demux/374 -> motor_to_central_differential/8  "Power_KW"
  Demux/375 -> motor_to_central_differential/9  "TCS_activity"
  Demux/376 -> motor_to_central_differential/10  "Theoretical_Power_KW"
  Demux/377 -> motor_to_central_differential/11  "torque"
  motor_to_clutch/1 -> OutputBus/42  "motor_to_clutch"
  Demux/378 -> motor_to_clutch/1  "clutch_inputplate_alpha"
  Demux/379 -> motor_to_clutch/2  "clutch_inputplate_angle"
  Demux/380 -> motor_to_clutch/3  "clutch_inputplate_omega"
  Demux/381 -> motor_to_clutch/4  "effective_throttle"
  Demux/382 -> motor_to_clutch/5  "engine_rpm"
  Demux/383 -> motor_to_clutch/6  "Max_Engine_torque"
  Demux/384 -> motor_to_clutch/7  "Min_engine_torque"
  Demux/385 -> motor_to_clutch/8  "Power_KW"
  Demux/386 -> motor_to_clutch/9  "TCS_activity"
  Demux/387 -> motor_to_clutch/10  "Theoretical_Power_KW"
  Demux/388 -> motor_to_clutch/11  "torque"
  motor_to_front_differential/1 -> OutputBus/43  "motor_to_front_differential"
  Demux/389 -> motor_to_front_differential/1  "differential_inputshaft_alpha"
  Demux/390 -> motor_to_front_differential/2  "differential_inputshaft_angle"
  Demux/391 -> motor_to_front_differential/3  "differential_inputshaft_omega"
  Demux/392 -> motor_to_front_differential/4  "effective_throttle"
  Demux/393 -> motor_to_front_differential/5  "engine_rpm"
  Demux/394 -> motor_to_front_differential/6  "Max_Engine_torque"
  Demux/395 -> motor_to_front_differential/7  "Min_engine_torque"
  Demux/396 -> motor_to_front_differential/8  "Power_KW"
  Demux/397 -> motor_to_front_differential/9  "TCS_activity"
  Demux/398 -> motor_to_front_differential/10  "Theoretical_Power_KW"
  Demux/399 -> motor_to_front_differential/11  "torque"
  motor_to_front_left_wheel/1 -> OutputBus/44  "motor_to_front_left_wheel"
  Demux/400 -> motor_to_front_left_wheel/1  "effective_throttle"
  Demux/401 -> motor_to_front_left_wheel/2  "engine_rpm"
  Demux/402 -> motor_to_front_left_wheel/3  "Max_Engine_torque"
  Demux/403 -> motor_to_front_left_wheel/4  "Min_engine_torque"
  Demux/404 -> motor_to_front_left_wheel/5  "Power_KW"
  Demux/405 -> motor_to_front_left_wheel/6  "TCS_activity"
  Demux/406 -> motor_to_front_left_wheel/7  "Theoretical_Power_KW"
  Demux/407 -> motor_to_front_left_wheel/8  "torque"
  Demux/408 -> motor_to_front_left_wheel/9  "wheel_inputshaft_alpha"
  Demux/409 -> motor_to_front_left_wheel/10  "wheel_inputshaft_angle"
  Demux/410 -> motor_to_front_left_wheel/11  "wheel_inputshaft_omega"
  motor_to_front_right_wheel/1 -> OutputBus/45  "motor_to_front_right_wheel"
  Demux/411 -> motor_to_front_right_wheel/1  "effective_throttle"
  Demux/412 -> motor_to_front_right_wheel/2  "engine_rpm"
  Demux/413 -> motor_to_front_right_wheel/3  "Max_Engine_torque"
  Demux/414 -> motor_to_front_right_wheel/4  "Min_engine_torque"
  Demux/415 -> motor_to_front_right_wheel/5  "Power_KW"
  Demux/416 -> motor_to_front_right_wheel/6  "TCS_activity"
  Demux/417 -> motor_to_front_right_wheel/7  "Theoretical_Power_KW"
  Demux/418 -> motor_to_front_right_wheel/8  "torque"
  Demux/419 -> motor_to_front_right_wheel/9  "wheel_inputshaft_alpha"
  Demux/420 -> motor_to_front_right_wheel/10  "wheel_inputshaft_angle"
  Demux/421 -> motor_to_front_right_wheel/11  "wheel_inputshaft_omega"
  motor_to_gearbox/1 -> OutputBus/46  "motor_to_gearbox"
  Demux/422 -> motor_to_gearbox/1  "effective_throttle"
  Demux/423 -> motor_to_gearbox/2  "engine_rpm"
  Demux/424 -> motor_to_gearbox/3  "gearbox_inputplate_alpha"
  Demux/425 -> motor_to_gearbox/4  "gearbox_inputplate_angle"
  Demux/426 -> motor_to_gearbox/5  "gearbox_inputplate_omega"
  Demux/427 -> motor_to_gearbox/6  "Max_Engine_torque"
  Demux/428 -> motor_to_gearbox/7  "Min_engine_torque"
  Demux/429 -> motor_to_gearbox/8  "Power_KW"
  Demux/430 -> motor_to_gearbox/9  "TCS_activity"
  Demux/431 -> motor_to_gearbox/10  "Theoretical_Power_KW"
  Demux/432 -> motor_to_gearbox/11  "torque"
  motor_to_rear_differential/1 -> OutputBus/47  "motor_to_rear_differential"
  Demux/433 -> motor_to_rear_differential/1  "differential_inputshaft_alpha"
  Demux/434 -> motor_to_rear_differential/2  "differential_inputshaft_angle"
  Demux/435 -> motor_to_rear_differential/3  "differential_inputshaft_omega"
  Demux/436 -> motor_to_rear_differential/4  "effective_throttle"
  Demux/437 -> motor_to_rear_differential/5  "engine_rpm"
  Demux/438 -> motor_to_rear_differential/6  "Max_Engine_torque"
  Demux/439 -> motor_to_rear_differential/7  "Min_engine_torque"
  Demux/440 -> motor_to_rear_differential/8  "Power_KW"
  Demux/441 -> motor_to_rear_differential/9  "TCS_activity"
  Demux/442 -> motor_to_rear_differential/10  "Theoretical_Power_KW"
  Demux/443 -> motor_to_rear_differential/11  "torque"
  motor_to_rear_left_wheel/1 -> OutputBus/48  "motor_to_rear_left_wheel"
  Demux/444 -> motor_to_rear_left_wheel/1  "effective_throttle"
  Demux/445 -> motor_to_rear_left_wheel/2  "engine_rpm"
  Demux/446 -> motor_to_rear_left_wheel/3  "Max_Engine_torque"
  Demux/447 -> motor_to_rear_left_wheel/4  "Min_engine_torque"
  Demux/448 -> motor_to_rear_left_wheel/5  "Power_KW"
  Demux/449 -> motor_to_rear_left_wheel/6  "TCS_activity"
  Demux/450 -> motor_to_rear_left_wheel/7  "Theoretical_Power_KW"
  Demux/451 -> motor_to_rear_left_wheel/8  "torque"
  Demux/452 -> motor_to_rear_left_wheel/9  "wheel_inputshaft_alpha"
  Demux/453 -> motor_to_rear_left_wheel/10  "wheel_inputshaft_angle"
  Demux/454 -> motor_to_rear_left_wheel/11  "wheel_inputshaft_omega"
  motor_to_rear_right_wheel/1 -> OutputBus/49  "motor_to_rear_right_wheel"
  Demux/455 -> motor_to_rear_right_wheel/1  "effective_throttle"
  Demux/456 -> motor_to_rear_right_wheel/2  "engine_rpm"
  Demux/457 -> motor_to_rear_right_wheel/3  "Max_Engine_torque"
  Demux/458 -> motor_to_rear_right_wheel/4  "Min_engine_torque"
  Demux/459 -> motor_to_rear_right_wheel/5  "Power_KW"
  Demux/460 -> motor_to_rear_right_wheel/6  "TCS_activity"
  Demux/461 -> motor_to_rear_right_wheel/7  "Theoretical_Power_KW"
  Demux/462 -> motor_to_rear_right_wheel/8  "torque"
  Demux/463 -> motor_to_rear_right_wheel/9  "wheel_inputshaft_alpha"
  Demux/464 -> motor_to_rear_right_wheel/10  "wheel_inputshaft_angle"
  Demux/465 -> motor_to_rear_right_wheel/11  "wheel_inputshaft_omega"
  nsl_ride_spring_data/1 -> OutputBus/50  "nsl_ride_spring_data"
  Demux/466 -> nsl_ride_spring_data/1  "displacement_front"
  Demux/467 -> nsl_ride_spring_data/2  "displacement_rear"
  Demux/468 -> nsl_ride_spring_data/3  "force_front"
  Demux/469 -> nsl_ride_spring_data/4  "force_rear"
  Demux/470 -> nsl_ride_spring_data/5  "velocity_front"
  Demux/471 -> nsl_ride_spring_data/6  "velocity_rear"
  nsr_ride_spring_data/1 -> OutputBus/51  "nsr_ride_spring_data"
  Demux/472 -> nsr_ride_spring_data/1  "displacement_front"
  Demux/473 -> nsr_ride_spring_data/2  "displacement_rear"
  Demux/474 -> nsr_ride_spring_data/3  "force_front"
  Demux/475 -> nsr_ride_spring_data/4  "force_rear"
  Demux/476 -> nsr_ride_spring_data/5  "velocity_front"
  Demux/477 -> nsr_ride_spring_data/6  "velocity_rear"
  nss_ride_spring_data/1 -> OutputBus/52  "nss_ride_spring_data"
  Demux/478 -> nss_ride_spring_data/1  "displacement_front"
  Demux/479 -> nss_ride_spring_data/2  "displacement_rear"
  Demux/480 -> nss_ride_spring_data/3  "force_at_wheel_front"
  Demux/481 -> nss_ride_spring_data/4  "force_at_wheel_rear"
  Demux/482 -> nss_ride_spring_data/5  "force_front"
  Demux/483 -> nss_ride_spring_data/6  "force_rear"
  Demux/484 -> nss_ride_spring_data/7  "PID_PH_At_Spring_front"
  Demux/485 -> nss_ride_spring_data/8  "PID_PH_At_Spring_rear"
  Demux/486 -> nss_ride_spring_data/9  "velocity_front"
  Demux/487 -> nss_ride_spring_data/10  "velocity_rear"
  Rebound_Bumper/1 -> OutputBus/53  "Rebound_Bumper"
  Force_At_Bumper1/1 -> Rebound_Bumper/1  "Force_At_Bumper"
  Demux/488 -> Force_At_Bumper1/1  "L1"
  Demux/489 -> Force_At_Bumper1/2  "L2"
  Demux/490 -> Force_At_Bumper1/3  "R1"
  Demux/491 -> Force_At_Bumper1/4  "R2"
  Force_At_Wheel3/1 -> Rebound_Bumper/2  "Force_At_Wheel"
  Demux/492 -> Force_At_Wheel3/1  "L1"
  Demux/493 -> Force_At_Wheel3/2  "L2"
  Demux/494 -> Force_At_Wheel3/3  "R1"
  Demux/495 -> Force_At_Wheel3/4  "R2"
  Jounce3/1 -> Rebound_Bumper/3  "Jounce"
  Demux/496 -> Jounce3/1  "L1"
  Demux/497 -> Jounce3/2  "L2"
  Demux/498 -> Jounce3/3  "R1"
  Demux/499 -> Jounce3/4  "R2"
  Jounce_Rate3/1 -> Rebound_Bumper/4  "Jounce_Rate"
  Demux/500 -> Jounce_Rate3/1  "L1"
  Demux/501 -> Jounce_Rate3/2  "L2"
  Demux/502 -> Jounce_Rate3/3  "R1"
  Demux/503 -> Jounce_Rate3/4  "R2"
  res_dmp_rebound_stop_data/1 -> OutputBus/54  "res_dmp_rebound_stop_data"
  Demux/504 -> res_dmp_rebound_stop_data/1  "displacement_front"
  Demux/505 -> res_dmp_rebound_stop_data/2  "displacement_rear"
  Demux/506 -> res_dmp_rebound_stop_data/3  "force_front"
  Demux/507 -> res_dmp_rebound_stop_data/4  "force_rear"
  Demux/508 -> res_dmp_rebound_stop_data/5  "velocity_front"
  Demux/509 -> res_dmp_rebound_stop_data/6  "velocity_rear"
  res_ins_rebound_stop_data/1 -> OutputBus/55  "res_ins_rebound_stop_data"
  Demux/510 -> res_ins_rebound_stop_data/1  "displacement_front"
  Demux/511 -> res_ins_rebound_stop_data/2  "displacement_rear"
  Demux/512 -> res_ins_rebound_stop_data/3  "force_front"
  Demux/513 -> res_ins_rebound_stop_data/4  "force_rear"
  Demux/514 -> res_ins_rebound_stop_data/5  "velocity_front"
  Demux/515 -> res_ins_rebound_stop_data/6  "velocity_rear"
  res_roll_dmp_rebound_stop_data/1 -> OutputBus/56  "res_roll_dmp_rebound_stop_data"
  Demux/516 -> res_roll_dmp_rebound_stop_data/1  "displacement_front"
  Demux/517 -> res_roll_dmp_rebound_stop_data/2  "displacement_rear"
  Demux/518 -> res_roll_dmp_rebound_stop_data/3  "force_front"
  Demux/519 -> res_roll_dmp_rebound_stop_data/4  "force_rear"
  Demux/520 -> res_roll_dmp_rebound_stop_data/5  "velocity_front"
  Demux/521 -> res_roll_dmp_rebound_stop_data/6  "velocity_rear"
  res_spr_rebound_stop_data/1 -> OutputBus/57  "res_spr_rebound_stop_data"
  Demux/522 -> res_spr_rebound_stop_data/1  "displacement_front"
  Demux/523 -> res_spr_rebound_stop_data/2  "displacement_rear"
  Demux/524 -> res_spr_rebound_stop_data/3  "force_front"
  Demux/525 -> res_spr_rebound_stop_data/4  "force_rear"
  Demux/526 -> res_spr_rebound_stop_data/5  "velocity_front"
  Demux/527 -> res_spr_rebound_stop_data/6  "velocity_rear"
  rhl_front_setup_sensor_data/1 -> OutputBus/58  "rhl_front_setup_sensor_data"
  Demux/528 -> rhl_front_setup_sensor_data/1  "ride_height"
  rhl_rear_setup_sensor_data/1 -> OutputBus/59  "rhl_rear_setup_sensor_data"
  Demux/529 -> rhl_rear_setup_sensor_data/1  "ride_height"
  rhr_front_setup_sensor_data/1 -> OutputBus/60  "rhr_front_setup_sensor_data"
  Demux/530 -> rhr_front_setup_sensor_data/1  "ride_height"
  rhr_rear_setup_sensor_data/1 -> OutputBus/61  "rhr_rear_setup_sensor_data"
  Demux/531 -> rhr_rear_setup_sensor_data/1  "ride_height"
  rhs_front_setup_sensor_data/1 -> OutputBus/62  "rhs_front_setup_sensor_data"
  Demux/532 -> rhs_front_setup_sensor_data/1  "ride_height"
  rhs_rear_setup_sensor_data/1 -> OutputBus/63  "rhs_rear_setup_sensor_data"
  Demux/533 -> rhs_rear_setup_sensor_data/1  "ride_height"
  Road/1 -> OutputBus/64  "Road"
  Contact_Flag/1 -> Road/1  "Contact_Flag"
  Demux/534 -> Contact_Flag/1  "L1"
  Demux/535 -> Contact_Flag/2  "L2"
  Demux/536 -> Contact_Flag/3  "R1"
  Demux/537 -> Contact_Flag/4  "R2"
  Contact_Patch_Global_X/1 -> Road/2  "Contact_Patch_Global_X"
  Demux/538 -> Contact_Patch_Global_X/1  "L1"
  Demux/539 -> Contact_Patch_Global_X/2  "L2"
  Demux/540 -> Contact_Patch_Global_X/3  "R1"
  Demux/541 -> Contact_Patch_Global_X/4  "R2"
  Contact_Patch_Global_Y/1 -> Road/3  "Contact_Patch_Global_Y"
  Demux/542 -> Contact_Patch_Global_Y/1  "L1"
  Demux/543 -> Contact_Patch_Global_Y/2  "L2"
  Demux/544 -> Contact_Patch_Global_Y/3  "R1"
  Demux/545 -> Contact_Patch_Global_Y/4  "R2"
  Contact_Patch_Global_Z/1 -> Road/4  "Contact_Patch_Global_Z"
  Demux/546 -> Contact_Patch_Global_Z/1  "L1"
  Demux/547 -> Contact_Patch_Global_Z/2  "L2"
  Demux/548 -> Contact_Patch_Global_Z/3  "R1"
  Demux/549 -> Contact_Patch_Global_Z/4  "R2"
  Off_Road_Flag/1 -> Road/5  "Off_Road_Flag"
  Demux/550 -> Off_Road_Flag/1  "L1"
  Demux/551 -> Off_Road_Flag/2  "L2"
  Demux/552 -> Off_Road_Flag/3  "R1"
  Demux/553 -> Off_Road_Flag/4  "R2"
  Sensor/1 -> OutputBus/65  "Sensor"
  Demux/554 -> Sensor/1  "AccX_gyro"
  Demux/555 -> Sensor/2  "AccY_gyro"
  Demux/556 -> Sensor/3  "Ax"
  Demux/557 -> Sensor/4  "Ax_Without_Gravity"
  Demux/558 -> Sensor/5  "Ay"
  Demux/559 -> Sensor/6  "Ay_Without_Gravity"
  Demux/560 -> Sensor/7  "Az"
  Demux/561 -> Sensor/8  "Az_Without_Gravity"
  Demux/562 -> Sensor/9  "Global_X"
  Demux/563 -> Sensor/10  "Global_Y"
  Demux/564 -> Sensor/11  "Global_Z"
  Demux/565 -> Sensor/12  "Vx"
  Demux/566 -> Sensor/13  "Vx_gyro"
  Demux/567 -> Sensor/14  "Vy"
  Demux/568 -> Sensor/15  "Vz"
  Demux/569 -> Sensor/16  "YawRate_gyro"
  Spring/1 -> OutputBus/66  "Spring"
  Aggregate_Force_At_Wheel/1 -> Spring/1  "Aggregate_Force_At_Wheel"
  Demux/570 -> Aggregate_Force_At_Wheel/1  "L1"
  Demux/571 -> Aggregate_Force_At_Wheel/2  "L2"
  Demux/572 -> Aggregate_Force_At_Wheel/3  "R1"
  Demux/573 -> Aggregate_Force_At_Wheel/4  "R2"
  Force_At_Spring/1 -> Spring/2  "Force_At_Spring"
  Demux/574 -> Force_At_Spring/1  "L1"
  Demux/575 -> Force_At_Spring/2  "L2"
  Demux/576 -> Force_At_Spring/3  "R1"
  Demux/577 -> Force_At_Spring/4  "R2"
  Force_At_Wheel4/1 -> Spring/3  "Force_At_Wheel"
  Demux/578 -> Force_At_Wheel4/1  "L1"
  Demux/579 -> Force_At_Wheel4/2  "L2"
  Demux/580 -> Force_At_Wheel4/3  "R1"
  Demux/581 -> Force_At_Wheel4/4  "R2"
  Force_Aux_At_Wheel/1 -> Spring/4  "Force_Aux_At_Wheel"
  Demux/582 -> Force_Aux_At_Wheel/1  "L1"
  Demux/583 -> Force_Aux_At_Wheel/2  "L2"
  Demux/584 -> Force_Aux_At_Wheel/3  "R1"
  Demux/585 -> Force_Aux_At_Wheel/4  "R2"
  Jounce4/1 -> Spring/5  "Jounce"
  Demux/586 -> Jounce4/1  "L1"
  Demux/587 -> Jounce4/2  "L2"
  Demux/588 -> Jounce4/3  "R1"
  Demux/589 -> Jounce4/4  "R2"
  Jounce_Acceleration2/1 -> Spring/6  "Jounce_Acceleration"
  Demux/590 -> Jounce_Acceleration2/1  "L1"
  Demux/591 -> Jounce_Acceleration2/2  "L2"
  Demux/592 -> Jounce_Acceleration2/3  "R1"
  Demux/593 -> Jounce_Acceleration2/4  "R2"
  Jounce_Rate4/1 -> Spring/7  "Jounce_Rate"
  Demux/594 -> Jounce_Rate4/1  "L1"
  Demux/595 -> Jounce_Rate4/2  "L2"
  Demux/596 -> Jounce_Rate4/3  "R1"
  Demux/597 -> Jounce_Rate4/4  "R2"
  PID_CW_At_Spring/1 -> Spring/8  "PID_CW_At_Spring"
  Demux/598 -> PID_CW_At_Spring/1  "L1"
  Demux/599 -> PID_CW_At_Spring/2  "L2"
  Demux/600 -> PID_CW_At_Spring/3  "R1"
  Demux/601 -> PID_CW_At_Spring/4  "R2"
  PID_PH_At_Spring/1 -> Spring/9  "PID_PH_At_Spring"
  Demux/602 -> PID_PH_At_Spring/1  "L1"
  Demux/603 -> PID_PH_At_Spring/2  "L2"
  Demux/604 -> PID_PH_At_Spring/3  "R1"
  Demux/605 -> PID_PH_At_Spring/4  "R2"
  PID_RH_At_Spring/1 -> Spring/10  "PID_RH_At_Spring"
  Demux/606 -> PID_RH_At_Spring/1  "L1"
  Demux/607 -> PID_RH_At_Spring/2  "L2"
  Demux/608 -> PID_RH_At_Spring/3  "R1"
  Demux/609 -> PID_RH_At_Spring/4  "R2"
  Steering_System/1 -> OutputBus/67  "Steering_System"
  Demux/610 -> Steering_System/1  "DriveSim_Steering_Feedback_Torque"
  Demux/611 -> Steering_System/2  "Rack_displacement"
  Demux/612 -> Steering_System/3  "Rack_Force"
  Demux/613 -> Steering_System/4  "Steering_column_deformation"
  Demux/614 -> Steering_System/5  "Steering_Wheel_Torque"
  TieRod_Force_Left/1 -> Steering_System/6  "TieRod_Force_Left"
  Demux/615 -> TieRod_Force_Left/1  "X"
  Demux/616 -> TieRod_Force_Left/2  "Y"
  Demux/617 -> TieRod_Force_Left/3  "Z"
  TieRod_Force_Right/1 -> Steering_System/7  "TieRod_Force_Right"
  Demux/618 -> TieRod_Force_Right/1  "X"
  Demux/619 -> TieRod_Force_Right/2  "Y"
  Demux/620 -> TieRod_Force_Right/3  "Z"
  Suspension/1 -> OutputBus/68  "Suspension"
  Auxiliary_Roll_deformation_at_element/1 -> Suspension/1  "Auxiliary_Roll_deformation_at_element"
  Demux/621 -> Auxiliary_Roll_deformation_at_element/1  "SUSP1"
  Demux/622 -> Auxiliary_Roll_deformation_at_element/2  "SUSP2"
  Auxiliary_Roll_Force/1 -> Suspension/2  "Auxiliary_Roll_Force"
  Demux/623 -> Auxiliary_Roll_Force/1  "SUSP_L1"
  Demux/624 -> Auxiliary_Roll_Force/2  "SUSP_L2"
  Demux/625 -> Auxiliary_Roll_Force/3  "SUSP_R1"
  Demux/626 -> Auxiliary_Roll_Force/4  "SUSP_R2"
  Auxiliary_Roll_Force_at_element/1 -> Suspension/3  "Auxiliary_Roll_Force_at_element"
  Demux/627 -> Auxiliary_Roll_Force_at_element/1  "SUSP1"
  Demux/628 -> Auxiliary_Roll_Force_at_element/2  "SUSP2"
  base_acceleration/1 -> Suspension/4  "base_acceleration"
  Demux/629 -> base_acceleration/1  "L1"
  Demux/630 -> base_acceleration/2  "L2"
  Demux/631 -> base_acceleration/3  "R1"
  Demux/632 -> base_acceleration/4  "R2"
  base_deformation/1 -> Suspension/5  "base_deformation"
  Demux/633 -> base_deformation/1  "L1"
  Demux/634 -> base_deformation/2  "L2"
  Demux/635 -> base_deformation/3  "R1"
  Demux/636 -> base_deformation/4  "R2"
  base_velocity/1 -> Suspension/6  "base_velocity"
  Demux/637 -> base_velocity/1  "L1"
  Demux/638 -> base_velocity/2  "L2"
  Demux/639 -> base_velocity/3  "R1"
  Demux/640 -> base_velocity/4  "R2"
  Inst_Stiff_Deflection/1 -> Suspension/7  "Inst_Stiff_Deflection"
  Demux/641 -> Inst_Stiff_Deflection/1  "front_left"
  Demux/642 -> Inst_Stiff_Deflection/2  "front_right"
  Demux/643 -> Inst_Stiff_Deflection/3  "rear_left"
  Demux/644 -> Inst_Stiff_Deflection/4  "rear_right"
  Inst_Stiff_Force/1 -> Suspension/8  "Inst_Stiff_Force"
  Demux/645 -> Inst_Stiff_Force/1  "front_left"
  Demux/646 -> Inst_Stiff_Force/2  "front_right"
  Demux/647 -> Inst_Stiff_Force/3  "rear_left"
  Demux/648 -> Inst_Stiff_Force/4  "rear_right"
  Jounce5/1 -> Suspension/9  "Jounce"
  Demux/649 -> Jounce5/1  "L1"
  Demux/650 -> Jounce5/2  "L2"
  Demux/651 -> Jounce5/3  "R1"
  Demux/652 -> Jounce5/4  "R2"
  Jounce_Acceleration3/1 -> Suspension/10  "Jounce_Acceleration"
  Demux/653 -> Jounce_Acceleration3/1  "L1"
  Demux/654 -> Jounce_Acceleration3/2  "L2"
  Demux/655 -> Jounce_Acceleration3/3  "R1"
  Demux/656 -> Jounce_Acceleration3/4  "R2"
  Jounce_Rate5/1 -> Suspension/11  "Jounce_Rate"
  Demux/657 -> Jounce_Rate5/1  "L1"
  Demux/658 -> Jounce_Rate5/2  "L2"
  Demux/659 -> Jounce_Rate5/3  "R1"
  Demux/660 -> Jounce_Rate5/4  "R2"
  Kingpin_Moment/1 -> Suspension/12  "Kingpin_Moment"
  Demux/661 -> Kingpin_Moment/1  "SUSP1"
  Roll/1 -> Suspension/13  "Roll"
  Demux/662 -> Roll/1  "SUSP1"
  Demux/663 -> Roll/2  "SUSP2"
  Roll_Center_Height/1 -> Suspension/14  "Roll_Center_Height"
  Demux/664 -> Roll_Center_Height/1  "front"
  Demux/665 -> Roll_Center_Height/2  "rear"
  Roll_Center_Lateral_Displacement/1 -> Suspension/15  "Roll_Center_Lateral_Displacement"
  Demux/666 -> Roll_Center_Lateral_Displacement/1  "front"
  Demux/667 -> Roll_Center_Lateral_Displacement/2  "rear"
  Steering_Instant_Axis_Rotation/1 -> Suspension/16  "Steering_Instant_Axis_Rotation"
  Demux/668 -> Steering_Instant_Axis_Rotation/1  "L1"
  Demux/669 -> Steering_Instant_Axis_Rotation/2  "R1"
  System/1 -> OutputBus/69  "System"
  Demux/670 -> System/1  "Angular_Acceleration_Norm"
  Demux/671 -> System/2  "Angular_Speed_Norm"
  Demux/672 -> System/3  "Testrig_MMM_Fx"
  Demux/673 -> System/4  "Testrig_MMM_Fy"
  Demux/674 -> System/5  "Testrig_MMM_Mz"
  Demux/675 -> System/6  "Testrig_MMM_xd"
  Demux/676 -> System/7  "Testrig_MMM_xi"
  Demux/677 -> System/8  "Testrig_MMM_xp"
  Demux/678 -> System/9  "Testrig_MMM_yawd"
  Demux/679 -> System/10  "Testrig_MMM_yawi"
  Demux/680 -> System/11  "Testrig_MMM_yawp"
  Demux/681 -> System/12  "Testrig_MMM_yd"
  Demux/682 -> System/13  "Testrig_MMM_yi"
  Demux/683 -> System/14  "Testrig_MMM_yp"
  Demux/684 -> System/15  "Translational_Acceleration_Norm"
  Demux/685 -> System/16  "Translational_Speed_Norm"
  Demux/1298 -> System/17  "Solver_Status"
  System_Mass_Center/1 -> OutputBus/70  "System_Mass_Center"
  Demux/686 -> System_Mass_Center/1  "Global_Ax"
  Demux/687 -> System_Mass_Center/2  "Global_Ay"
  Demux/688 -> System_Mass_Center/3  "Global_Az"
  Demux/689 -> System_Mass_Center/4  "Global_Vx"
  Demux/690 -> System_Mass_Center/5  "Global_Vy"
  Demux/691 -> System_Mass_Center/6  "Global_Vz"
  Demux/692 -> System_Mass_Center/7  "Global_X"
  Demux/693 -> System_Mass_Center/8  "Global_Y"
  Demux/694 -> System_Mass_Center/9  "Global_Z"
  Demux/695 -> System_Mass_Center/10  "Normal_Acceleration"
  Demux/696 -> System_Mass_Center/11  "Path_Curvature"
  Demux/697 -> System_Mass_Center/12  "Speed"
  Demux/698 -> System_Mass_Center/13  "Tangential_Acceleration"
  til_wheel_tire_forces/1 -> OutputBus/71  "til_wheel_tire_forces"
  Demux/699 -> til_wheel_tire_forces/1  "aligning_torque_front"
  Demux/700 -> til_wheel_tire_forces/2  "aligning_torque_rear"
  Demux/701 -> til_wheel_tire_forces/3  "aligning_torque_twin_rear"
  Demux/702 -> til_wheel_tire_forces/4  "lateral_front"
  Demux/703 -> til_wheel_tire_forces/5  "lateral_rear"
  Demux/704 -> til_wheel_tire_forces/6  "lateral_twin_rear"
  Demux/705 -> til_wheel_tire_forces/7  "longitudinal_front"
  Demux/706 -> til_wheel_tire_forces/8  "longitudinal_rear"
  Demux/707 -> til_wheel_tire_forces/9  "longitudinal_twin_rear"
  Demux/708 -> til_wheel_tire_forces/10  "normal_front"
  Demux/709 -> til_wheel_tire_forces/11  "normal_rear"
  Demux/710 -> til_wheel_tire_forces/12  "normal_twin_rear"
  Demux/711 -> til_wheel_tire_forces/13  "overturning_moment_front"
  Demux/712 -> til_wheel_tire_forces/14  "overturning_moment_rear"
  Demux/713 -> til_wheel_tire_forces/15  "overturning_moment_twin_rear"
  Demux/714 -> til_wheel_tire_forces/16  "rolling_resistance_front"
  Demux/715 -> til_wheel_tire_forces/17  "rolling_resistance_rear"
  Demux/716 -> til_wheel_tire_forces/18  "rolling_resistance_twin_rear"
  til_wheel_tire_kinematics/1 -> OutputBus/72  "til_wheel_tire_kinematics"
  Demux/717 -> til_wheel_tire_kinematics/1  "inclination_angle_front"
  Demux/718 -> til_wheel_tire_kinematics/2  "inclination_angle_rear"
  Demux/719 -> til_wheel_tire_kinematics/3  "inclination_angle_twin_rear"
  Demux/720 -> til_wheel_tire_kinematics/4  "lateral_slip_front"
  Demux/721 -> til_wheel_tire_kinematics/5  "lateral_slip_rear"
  Demux/722 -> til_wheel_tire_kinematics/6  "lateral_slip_twin_rear"
  Demux/723 -> til_wheel_tire_kinematics/7  "longitudinal_slip_front"
  Demux/724 -> til_wheel_tire_kinematics/8  "longitudinal_slip_rear"
  Demux/725 -> til_wheel_tire_kinematics/9  "longitudinal_slip_twin_rear"
  til_wheel_tire_rolling_states/1 -> OutputBus/73  "til_wheel_tire_rolling_states"
  Demux/726 -> til_wheel_tire_rolling_states/1  "omega_actual_front"
  Demux/727 -> til_wheel_tire_rolling_states/2  "omega_actual_rear"
  Demux/728 -> til_wheel_tire_rolling_states/3  "omega_actual_twin_rear"
  Demux/729 -> til_wheel_tire_rolling_states/4  "omega_free_front"
  Demux/730 -> til_wheel_tire_rolling_states/5  "omega_free_rear"
  Demux/731 -> til_wheel_tire_rolling_states/6  "omega_free_twin_rear"
  Demux/732 -> til_wheel_tire_rolling_states/7  "rolling_radius_front"
  Demux/733 -> til_wheel_tire_rolling_states/8  "rolling_radius_rear"
  Demux/734 -> til_wheel_tire_rolling_states/9  "rolling_radius_twin_rear"
  Tire/1 -> OutputBus/74  "Tire"
  Actual_Tread_Speed/1 -> Tire/1  "Actual_Tread_Speed"
  Demux/735 -> Actual_Tread_Speed/1  "L1"
  Demux/736 -> Actual_Tread_Speed/2  "L2"
  Demux/737 -> Actual_Tread_Speed/3  "R1"
  Demux/738 -> Actual_Tread_Speed/4  "R2"
  Contact_Patch_Global_X1/1 -> Tire/2  "Contact_Patch_Global_X"
  Demux/739 -> Contact_Patch_Global_X1/1  "L1"
  Demux/740 -> Contact_Patch_Global_X1/2  "L2"
  Demux/741 -> Contact_Patch_Global_X1/3  "R1"
  Demux/742 -> Contact_Patch_Global_X1/4  "R2"
  Contact_Patch_Global_Y1/1 -> Tire/3  "Contact_Patch_Global_Y"
  Demux/743 -> Contact_Patch_Global_Y1/1  "L1"
  Demux/744 -> Contact_Patch_Global_Y1/2  "L2"
  Demux/745 -> Contact_Patch_Global_Y1/3  "R1"
  Demux/746 -> Contact_Patch_Global_Y1/4  "R2"
  Contact_Patch_Global_Z1/1 -> Tire/4  "Contact_Patch_Global_Z"
  Demux/747 -> Contact_Patch_Global_Z1/1  "L1"
  Demux/748 -> Contact_Patch_Global_Z1/2  "L2"
  Demux/749 -> Contact_Patch_Global_Z1/3  "R1"
  Demux/750 -> Contact_Patch_Global_Z1/4  "R2"
  Contact_Patch_Normal_X/1 -> Tire/5  "Contact_Patch_Normal_X"
  Demux/751 -> Contact_Patch_Normal_X/1  "L1"
  Demux/752 -> Contact_Patch_Normal_X/2  "L2"
  Demux/753 -> Contact_Patch_Normal_X/3  "R1"
  Demux/754 -> Contact_Patch_Normal_X/4  "R2"
  Contact_Patch_Normal_Y/1 -> Tire/6  "Contact_Patch_Normal_Y"
  Demux/755 -> Contact_Patch_Normal_Y/1  "L1"
  Demux/756 -> Contact_Patch_Normal_Y/2  "L2"
  Demux/757 -> Contact_Patch_Normal_Y/3  "R1"
  Demux/758 -> Contact_Patch_Normal_Y/4  "R2"
  Contact_Patch_Normal_Z/1 -> Tire/7  "Contact_Patch_Normal_Z"
  Demux/759 -> Contact_Patch_Normal_Z/1  "L1"
  Demux/760 -> Contact_Patch_Normal_Z/2  "L2"
  Demux/761 -> Contact_Patch_Normal_Z/3  "R1"
  Demux/762 -> Contact_Patch_Normal_Z/4  "R2"
  Effective_Closing_Speed/1 -> Tire/8  "Effective_Closing_Speed"
  Demux/763 -> Effective_Closing_Speed/1  "L1"
  Demux/764 -> Effective_Closing_Speed/2  "L2"
  Demux/765 -> Effective_Closing_Speed/3  "R1"
  Demux/766 -> Effective_Closing_Speed/4  "R2"
  Effective_Penetration/1 -> Tire/9  "Effective_Penetration"
  Demux/767 -> Effective_Penetration/1  "L1"
  Demux/768 -> Effective_Penetration/2  "L2"
  Demux/769 -> Effective_Penetration/3  "R1"
  Demux/770 -> Effective_Penetration/4  "R2"
  Effective_Rolling_Radius/1 -> Tire/10  "Effective_Rolling_Radius"
  Demux/771 -> Effective_Rolling_Radius/1  "L1"
  Demux/772 -> Effective_Rolling_Radius/2  "L2"
  Demux/773 -> Effective_Rolling_Radius/3  "R1"
  Demux/774 -> Effective_Rolling_Radius/4  "R2"
  Equivalent_Tread_Speed/1 -> Tire/11  "Equivalent_Tread_Speed"
  Demux/775 -> Equivalent_Tread_Speed/1  "L1"
  Demux/776 -> Equivalent_Tread_Speed/2  "L2"
  Demux/777 -> Equivalent_Tread_Speed/3  "R1"
  Demux/778 -> Equivalent_Tread_Speed/4  "R2"
  External_Friction_Scale_Factor/1 -> Tire/12  "External_Friction_Scale_Factor"
  Demux/779 -> External_Friction_Scale_Factor/1  "L1"
  Demux/780 -> External_Friction_Scale_Factor/2  "L2"
  Demux/781 -> External_Friction_Scale_Factor/3  "R1"
  Demux/782 -> External_Friction_Scale_Factor/4  "R2"
  Ground_Surface_Contact_Patch_Vx/1 -> Tire/13  "Ground_Surface_Contact_Patch_Vx"
  Demux/783 -> Ground_Surface_Contact_Patch_Vx/1  "L1"
  Demux/784 -> Ground_Surface_Contact_Patch_Vx/2  "L2"
  Demux/785 -> Ground_Surface_Contact_Patch_Vx/3  "R1"
  Demux/786 -> Ground_Surface_Contact_Patch_Vx/4  "R2"
  Ground_Surface_Contact_Patch_Vy/1 -> Tire/14  "Ground_Surface_Contact_Patch_Vy"
  Demux/787 -> Ground_Surface_Contact_Patch_Vy/1  "L1"
  Demux/788 -> Ground_Surface_Contact_Patch_Vy/2  "L2"
  Demux/789 -> Ground_Surface_Contact_Patch_Vy/3  "R1"
  Demux/790 -> Ground_Surface_Contact_Patch_Vy/4  "R2"
  Ground_Surface_Force_X/1 -> Tire/15  "Ground_Surface_Force_X"
  Demux/791 -> Ground_Surface_Force_X/1  "L1"
  Demux/792 -> Ground_Surface_Force_X/2  "L2"
  Demux/793 -> Ground_Surface_Force_X/3  "R1"
  Demux/794 -> Ground_Surface_Force_X/4  "R2"
  Ground_Surface_Force_Y/1 -> Tire/16  "Ground_Surface_Force_Y"
  Demux/795 -> Ground_Surface_Force_Y/1  "L1"
  Demux/796 -> Ground_Surface_Force_Y/2  "L2"
  Demux/797 -> Ground_Surface_Force_Y/3  "R1"
  Demux/798 -> Ground_Surface_Force_Y/4  "R2"
  Ground_Surface_Force_Z/1 -> Tire/17  "Ground_Surface_Force_Z"
  Demux/799 -> Ground_Surface_Force_Z/1  "L1"
  Demux/800 -> Ground_Surface_Force_Z/2  "L2"
  Demux/801 -> Ground_Surface_Force_Z/3  "R1"
  Demux/802 -> Ground_Surface_Force_Z/4  "R2"
  Ground_Surface_Gyroscopic_Moment/1 -> Tire/18  "Ground_Surface_Gyroscopic_Moment"
  Demux/803 -> Ground_Surface_Gyroscopic_Moment/1  "L1"
  Demux/804 -> Ground_Surface_Gyroscopic_Moment/2  "L2"
  Demux/805 -> Ground_Surface_Gyroscopic_Moment/3  "R1"
  Demux/806 -> Ground_Surface_Gyroscopic_Moment/4  "R2"
  Ground_Surface_Kappa_Fy/1 -> Tire/19  "Ground_Surface_Kappa_Fy"
  Demux/807 -> Ground_Surface_Kappa_Fy/1  "L1"
  Demux/808 -> Ground_Surface_Kappa_Fy/2  "L2"
  Demux/809 -> Ground_Surface_Kappa_Fy/3  "R1"
  Demux/810 -> Ground_Surface_Kappa_Fy/4  "R2"
  Ground_Surface_Moment_X/1 -> Tire/20  "Ground_Surface_Moment_X"
  Demux/811 -> Ground_Surface_Moment_X/1  "L1"
  Demux/812 -> Ground_Surface_Moment_X/2  "L2"
  Demux/813 -> Ground_Surface_Moment_X/3  "R1"
  Demux/814 -> Ground_Surface_Moment_X/4  "R2"
  Ground_Surface_Moment_Y/1 -> Tire/21  "Ground_Surface_Moment_Y"
  Demux/815 -> Ground_Surface_Moment_Y/1  "L1"
  Demux/816 -> Ground_Surface_Moment_Y/2  "L2"
  Demux/817 -> Ground_Surface_Moment_Y/3  "R1"
  Demux/818 -> Ground_Surface_Moment_Y/4  "R2"
  Ground_Surface_Moment_Z/1 -> Tire/22  "Ground_Surface_Moment_Z"
  Demux/819 -> Ground_Surface_Moment_Z/1  "L1"
  Demux/820 -> Ground_Surface_Moment_Z/2  "L2"
  Demux/821 -> Ground_Surface_Moment_Z/3  "R1"
  Demux/822 -> Ground_Surface_Moment_Z/4  "R2"
  Ground_Surface_Peak_Friction_X/1 -> Tire/23  "Ground_Surface_Peak_Friction_X"
  Demux/823 -> Ground_Surface_Peak_Friction_X/1  "L1"
  Demux/824 -> Ground_Surface_Peak_Friction_X/2  "L2"
  Demux/825 -> Ground_Surface_Peak_Friction_X/3  "R1"
  Demux/826 -> Ground_Surface_Peak_Friction_X/4  "R2"
  Ground_Surface_Peak_Friction_Y/1 -> Tire/24  "Ground_Surface_Peak_Friction_Y"
  Demux/827 -> Ground_Surface_Peak_Friction_Y/1  "L1"
  Demux/828 -> Ground_Surface_Peak_Friction_Y/2  "L2"
  Demux/829 -> Ground_Surface_Peak_Friction_Y/3  "R1"
  Demux/830 -> Ground_Surface_Peak_Friction_Y/4  "R2"
  Ground_Surface_Residual_Torque/1 -> Tire/25  "Ground_Surface_Residual_Torque"
  Demux/831 -> Ground_Surface_Residual_Torque/1  "L1"
  Demux/832 -> Ground_Surface_Residual_Torque/2  "L2"
  Demux/833 -> Ground_Surface_Residual_Torque/3  "R1"
  Demux/834 -> Ground_Surface_Residual_Torque/4  "R2"
  Hub_Carrier_Force_Global_X/1 -> Tire/26  "Hub_Carrier_Force_Global_X"
  Demux/835 -> Hub_Carrier_Force_Global_X/1  "L1"
  Demux/836 -> Hub_Carrier_Force_Global_X/2  "L2"
  Demux/837 -> Hub_Carrier_Force_Global_X/3  "R1"
  Demux/838 -> Hub_Carrier_Force_Global_X/4  "R2"
  Hub_Carrier_Force_Global_Y/1 -> Tire/27  "Hub_Carrier_Force_Global_Y"
  Demux/839 -> Hub_Carrier_Force_Global_Y/1  "L1"
  Demux/840 -> Hub_Carrier_Force_Global_Y/2  "L2"
  Demux/841 -> Hub_Carrier_Force_Global_Y/3  "R1"
  Demux/842 -> Hub_Carrier_Force_Global_Y/4  "R2"
  Hub_Carrier_Force_Global_Z/1 -> Tire/28  "Hub_Carrier_Force_Global_Z"
  Demux/843 -> Hub_Carrier_Force_Global_Z/1  "L1"
  Demux/844 -> Hub_Carrier_Force_Global_Z/2  "L2"
  Demux/845 -> Hub_Carrier_Force_Global_Z/3  "R1"
  Demux/846 -> Hub_Carrier_Force_Global_Z/4  "R2"
  Hub_Carrier_Force_Local_X/1 -> Tire/29  "Hub_Carrier_Force_Local_X"
  Demux/847 -> Hub_Carrier_Force_Local_X/1  "L1"
  Demux/848 -> Hub_Carrier_Force_Local_X/2  "L2"
  Demux/849 -> Hub_Carrier_Force_Local_X/3  "R1"
  Demux/850 -> Hub_Carrier_Force_Local_X/4  "R2"
  Hub_Carrier_Force_Local_Y/1 -> Tire/30  "Hub_Carrier_Force_Local_Y"
  Demux/851 -> Hub_Carrier_Force_Local_Y/1  "L1"
  Demux/852 -> Hub_Carrier_Force_Local_Y/2  "L2"
  Demux/853 -> Hub_Carrier_Force_Local_Y/3  "R1"
  Demux/854 -> Hub_Carrier_Force_Local_Y/4  "R2"
  Hub_Carrier_Force_Local_Z/1 -> Tire/31  "Hub_Carrier_Force_Local_Z"
  Demux/855 -> Hub_Carrier_Force_Local_Z/1  "L1"
  Demux/856 -> Hub_Carrier_Force_Local_Z/2  "L2"
  Demux/857 -> Hub_Carrier_Force_Local_Z/3  "R1"
  Demux/858 -> Hub_Carrier_Force_Local_Z/4  "R2"
  Hub_Carrier_Moment_Global_X/1 -> Tire/32  "Hub_Carrier_Moment_Global_X"
  Demux/859 -> Hub_Carrier_Moment_Global_X/1  "L1"
  Demux/860 -> Hub_Carrier_Moment_Global_X/2  "L2"
  Demux/861 -> Hub_Carrier_Moment_Global_X/3  "R1"
  Demux/862 -> Hub_Carrier_Moment_Global_X/4  "R2"
  Hub_Carrier_Moment_Global_Y/1 -> Tire/33  "Hub_Carrier_Moment_Global_Y"
  Demux/863 -> Hub_Carrier_Moment_Global_Y/1  "L1"
  Demux/864 -> Hub_Carrier_Moment_Global_Y/2  "L2"
  Demux/865 -> Hub_Carrier_Moment_Global_Y/3  "R1"
  Demux/866 -> Hub_Carrier_Moment_Global_Y/4  "R2"
  Hub_Carrier_Moment_Global_Z/1 -> Tire/34  "Hub_Carrier_Moment_Global_Z"
  Demux/867 -> Hub_Carrier_Moment_Global_Z/1  "L1"
  Demux/868 -> Hub_Carrier_Moment_Global_Z/2  "L2"
  Demux/869 -> Hub_Carrier_Moment_Global_Z/3  "R1"
  Demux/870 -> Hub_Carrier_Moment_Global_Z/4  "R2"
  Hub_Carrier_Moment_Local_X/1 -> Tire/35  "Hub_Carrier_Moment_Local_X"
  Demux/871 -> Hub_Carrier_Moment_Local_X/1  "L1"
  Demux/872 -> Hub_Carrier_Moment_Local_X/2  "L2"
  Demux/873 -> Hub_Carrier_Moment_Local_X/3  "R1"
  Demux/874 -> Hub_Carrier_Moment_Local_X/4  "R2"
  Hub_Carrier_Moment_Local_Y/1 -> Tire/36  "Hub_Carrier_Moment_Local_Y"
  Demux/875 -> Hub_Carrier_Moment_Local_Y/1  "L1"
  Demux/876 -> Hub_Carrier_Moment_Local_Y/2  "L2"
  Demux/877 -> Hub_Carrier_Moment_Local_Y/3  "R1"
  Demux/878 -> Hub_Carrier_Moment_Local_Y/4  "R2"
  Hub_Carrier_Moment_Local_Z/1 -> Tire/37  "Hub_Carrier_Moment_Local_Z"
  Demux/879 -> Hub_Carrier_Moment_Local_Z/1  "L1"
  Demux/880 -> Hub_Carrier_Moment_Local_Z/2  "L2"
  Demux/881 -> Hub_Carrier_Moment_Local_Z/3  "R1"
  Demux/882 -> Hub_Carrier_Moment_Local_Z/4  "R2"
  Lateral_Relaxation_Length/1 -> Tire/38  "Lateral_Relaxation_Length"
  Demux/883 -> Lateral_Relaxation_Length/1  "L1"
  Demux/884 -> Lateral_Relaxation_Length/2  "L2"
  Demux/885 -> Lateral_Relaxation_Length/3  "R1"
  Demux/886 -> Lateral_Relaxation_Length/4  "R2"
  Lateral_Slip_Without_Lag/1 -> Tire/39  "Lateral_Slip_Without_Lag"
  Demux/887 -> Lateral_Slip_Without_Lag/1  "L1"
  Demux/888 -> Lateral_Slip_Without_Lag/2  "L2"
  Demux/889 -> Lateral_Slip_Without_Lag/3  "R1"
  Demux/890 -> Lateral_Slip_Without_Lag/4  "R2"
  Lateral_Slip_With_Lag/1 -> Tire/40  "Lateral_Slip_With_Lag"
  Demux/891 -> Lateral_Slip_With_Lag/1  "L1"
  Demux/892 -> Lateral_Slip_With_Lag/2  "L2"
  Demux/893 -> Lateral_Slip_With_Lag/3  "R1"
  Demux/894 -> Lateral_Slip_With_Lag/4  "R2"
  Loaded_Radius/1 -> Tire/41  "Loaded_Radius"
  Demux/895 -> Loaded_Radius/1  "L1"
  Demux/896 -> Loaded_Radius/2  "L2"
  Demux/897 -> Loaded_Radius/3  "R1"
  Demux/898 -> Loaded_Radius/4  "R2"
  Longitudinal_Relaxation_Length/1 -> Tire/42  "Longitudinal_Relaxation_Length"
  Demux/899 -> Longitudinal_Relaxation_Length/1  "L1"
  Demux/900 -> Longitudinal_Relaxation_Length/2  "L2"
  Demux/901 -> Longitudinal_Relaxation_Length/3  "R1"
  Demux/902 -> Longitudinal_Relaxation_Length/4  "R2"
  Longitudinal_Slip_Without_Lag/1 -> Tire/43  "Longitudinal_Slip_Without_Lag"
  Demux/903 -> Longitudinal_Slip_Without_Lag/1  "L1"
  Demux/904 -> Longitudinal_Slip_Without_Lag/2  "L2"
  Demux/905 -> Longitudinal_Slip_Without_Lag/3  "R1"
  Demux/906 -> Longitudinal_Slip_Without_Lag/4  "R2"
  Longitudinal_Slip_With_Lag/1 -> Tire/44  "Longitudinal_Slip_With_Lag"
  Demux/907 -> Longitudinal_Slip_With_Lag/1  "L1"
  Demux/908 -> Longitudinal_Slip_With_Lag/2  "L2"
  Demux/909 -> Longitudinal_Slip_With_Lag/3  "R1"
  Demux/910 -> Longitudinal_Slip_With_Lag/4  "R2"
  Moment_Arm_Of_Fx/1 -> Tire/45  "Moment_Arm_Of_Fx"
  Demux/911 -> Moment_Arm_Of_Fx/1  "L1"
  Demux/912 -> Moment_Arm_Of_Fx/2  "L2"
  Demux/913 -> Moment_Arm_Of_Fx/3  "R1"
  Demux/914 -> Moment_Arm_Of_Fx/4  "R2"
  Pneumatic_Trail/1 -> Tire/46  "Pneumatic_Trail"
  Demux/915 -> Pneumatic_Trail/1  "L1"
  Demux/916 -> Pneumatic_Trail/2  "L2"
  Demux/917 -> Pneumatic_Trail/3  "R1"
  Demux/918 -> Pneumatic_Trail/4  "R2"
  Pressure/1 -> Tire/47  "Pressure"
  Demux/919 -> Pressure/1  "L1"
  Demux/920 -> Pressure/2  "L2"
  Demux/921 -> Pressure/3  "R1"
  Demux/922 -> Pressure/4  "R2"
  Road_friction/1 -> Tire/48  "Road_friction"
  Demux/923 -> Road_friction/1  "L1"
  Demux/924 -> Road_friction/2  "L2"
  Demux/925 -> Road_friction/3  "R1"
  Demux/926 -> Road_friction/4  "R2"
  Temperature_1/1 -> Tire/49  "Temperature_1"
  Demux/927 -> Temperature_1/1  "L1"
  Demux/928 -> Temperature_1/2  "L2"
  Demux/929 -> Temperature_1/3  "R1"
  Demux/930 -> Temperature_1/4  "R2"
  Temperature_2/1 -> Tire/50  "Temperature_2"
  Demux/931 -> Temperature_2/1  "L1"
  Demux/932 -> Temperature_2/2  "L2"
  Demux/933 -> Temperature_2/3  "R1"
  Demux/934 -> Temperature_2/4  "R2"
  Temperature_3/1 -> Tire/51  "Temperature_3"
  Demux/935 -> Temperature_3/1  "L1"
  Demux/936 -> Temperature_3/2  "L2"
  Demux/937 -> Temperature_3/3  "R1"
  Demux/938 -> Temperature_3/4  "R2"
  User_Input_Contact_Patch_Global_Z_Perturbation/1 -> Tire/52  "User_Input_Contact_Patch_Global_Z_Perturbation"
  Demux/939 -> User_Input_Contact_Patch_Global_Z_Perturbation/1  "L1"
  Demux/940 -> User_Input_Contact_Patch_Global_Z_Perturbation/2  "L2"
  Demux/941 -> User_Input_Contact_Patch_Global_Z_Perturbation/3  "R1"
  Demux/942 -> User_Input_Contact_Patch_Global_Z_Perturbation/4  "R2"
  tir_wheel_tire_forces/1 -> OutputBus/75  "tir_wheel_tire_forces"
  Demux/943 -> tir_wheel_tire_forces/1  "aligning_torque_front"
  Demux/944 -> tir_wheel_tire_forces/2  "aligning_torque_rear"
  Demux/945 -> tir_wheel_tire_forces/3  "aligning_torque_twin_rear"
  Demux/946 -> tir_wheel_tire_forces/4  "lateral_front"
  Demux/947 -> tir_wheel_tire_forces/5  "lateral_rear"
  Demux/948 -> tir_wheel_tire_forces/6  "lateral_twin_rear"
  Demux/949 -> tir_wheel_tire_forces/7  "longitudinal_front"
  Demux/950 -> tir_wheel_tire_forces/8  "longitudinal_rear"
  Demux/951 -> tir_wheel_tire_forces/9  "longitudinal_twin_rear"
  Demux/952 -> tir_wheel_tire_forces/10  "normal_front"
  Demux/953 -> tir_wheel_tire_forces/11  "normal_rear"
  Demux/954 -> tir_wheel_tire_forces/12  "normal_twin_rear"
  Demux/955 -> tir_wheel_tire_forces/13  "overturning_moment_front"
  Demux/956 -> tir_wheel_tire_forces/14  "overturning_moment_rear"
  Demux/957 -> tir_wheel_tire_forces/15  "overturning_moment_twin_rear"
  Demux/958 -> tir_wheel_tire_forces/16  "rolling_resistance_front"
  Demux/959 -> tir_wheel_tire_forces/17  "rolling_resistance_rear"
  Demux/960 -> tir_wheel_tire_forces/18  "rolling_resistance_twin_rear"
  tir_wheel_tire_kinematics/1 -> OutputBus/76  "tir_wheel_tire_kinematics"
  Demux/961 -> tir_wheel_tire_kinematics/1  "inclination_angle_front"
  Demux/962 -> tir_wheel_tire_kinematics/2  "inclination_angle_rear"
  Demux/963 -> tir_wheel_tire_kinematics/3  "inclination_angle_twin_rear"
  Demux/964 -> tir_wheel_tire_kinematics/4  "lateral_slip_front"
  Demux/965 -> tir_wheel_tire_kinematics/5  "lateral_slip_rear"
  Demux/966 -> tir_wheel_tire_kinematics/6  "lateral_slip_twin_rear"
  Demux/967 -> tir_wheel_tire_kinematics/7  "longitudinal_slip_front"
  Demux/968 -> tir_wheel_tire_kinematics/8  "longitudinal_slip_rear"
  Demux/969 -> tir_wheel_tire_kinematics/9  "longitudinal_slip_twin_rear"
  tir_wheel_tire_rolling_states/1 -> OutputBus/77  "tir_wheel_tire_rolling_states"
  Demux/970 -> tir_wheel_tire_rolling_states/1  "omega_actual_front"
  Demux/971 -> tir_wheel_tire_rolling_states/2  "omega_actual_rear"
  Demux/972 -> tir_wheel_tire_rolling_states/3  "omega_actual_twin_rear"
  Demux/973 -> tir_wheel_tire_rolling_states/4  "omega_free_front"
  Demux/974 -> tir_wheel_tire_rolling_states/5  "omega_free_rear"
  Demux/975 -> tir_wheel_tire_rolling_states/6  "omega_free_twin_rear"
  Demux/976 -> tir_wheel_tire_rolling_states/7  "rolling_radius_front"
  Demux/977 -> tir_wheel_tire_rolling_states/8  "rolling_radius_rear"
  Demux/978 -> tir_wheel_tire_rolling_states/9  "rolling_radius_twin_rear"
  torque_converter/1 -> OutputBus/78  "torque_converter"
  Demux/979 -> torque_converter/1  "capacity_factor"
  Demux/980 -> torque_converter/2  "efficiency"
  Demux/981 -> torque_converter/3  "gearbox_inputshaft_alpha"
  Demux/982 -> torque_converter/4  "gearbox_inputshaft_angle"
  Demux/983 -> torque_converter/5  "gearbox_inputshaft_omega"
  Demux/984 -> torque_converter/6  "inputplate_torque"
  Demux/985 -> torque_converter/7  "speed_ratio"
  Demux/986 -> torque_converter/8  "torque"
  Demux/987 -> torque_converter/9  "torque_ratio"
  transmission/1 -> OutputBus/79  "transmission"
  Demux/988 -> transmission/1  "automatic_gearbox_shifting_mode"
  Demux/989 -> transmission/2  "clutch_outputplate_torque"
  Demux/990 -> transmission/3  "diff_central_inputshaft_alpha"
  Demux/991 -> transmission/4  "diff_central_inputshaft_angle"
  Demux/992 -> transmission/5  "diff_central_inputshaft_omega"
  Demux/993 -> transmission/6  "gear"
  Demux/994 -> transmission/7  "input_rpm"
  Demux/995 -> transmission/8  "output_rpm"
  Demux/996 -> transmission/9  "ratio"
  Demux/997 -> transmission/10  "torque"
  ues_third_spring_data/1 -> OutputBus/80  "ues_third_spring_data"
  Demux/998 -> ues_third_spring_data/1  "displacement_front"
  Demux/999 -> ues_third_spring_data/2  "displacement_rear"
  Demux/1000 -> ues_third_spring_data/3  "force_front"
  Demux/1001 -> ues_third_spring_data/4  "force_rear"
  Demux/1002 -> ues_third_spring_data/5  "velocity_front"
  Demux/1003 -> ues_third_spring_data/6  "velocity_rear"
  upright_accelerometer/1 -> OutputBus/81  "upright_accelerometer"
  Demux/1004 -> upright_accelerometer/1  "Z_left_front"
  Demux/1005 -> upright_accelerometer/2  "Z_left_rear"
  Demux/1006 -> upright_accelerometer/3  "Z_right_front"
  Demux/1007 -> upright_accelerometer/4  "Z_right_rear"
  Vehicle/1 -> OutputBus/82  "Vehicle"
  Demux/1008 -> Vehicle/1  "Body_Fixed_Alpha_X"
  Demux/1009 -> Vehicle/2  "Body_Fixed_Alpha_Y"
  Demux/1010 -> Vehicle/3  "Body_Fixed_Alpha_Z"
  Demux/1011 -> Vehicle/4  "Body_Fixed_Omega_X"
  Demux/1012 -> Vehicle/5  "Body_Fixed_Omega_Y"
  Demux/1013 -> Vehicle/6  "Body_Fixed_Omega_Z"
  Demux/1014 -> Vehicle/7  "CM_Body_Fixed_Ax"
  Demux/1015 -> Vehicle/8  "CM_Body_Fixed_Ay"
  Demux/1016 -> Vehicle/9  "CM_Body_Fixed_Az"
  Demux/1017 -> Vehicle/10  "CM_Body_Fixed_Vx"
  Demux/1018 -> Vehicle/11  "CM_Body_Fixed_Vy"
  Demux/1019 -> Vehicle/12  "CM_Body_Fixed_Vz"
  Demux/1020 -> Vehicle/13  "CM_Global_And_Tracking_Az"
  Demux/1021 -> Vehicle/14  "CM_Global_And_Tracking_Vz"
  Demux/1022 -> Vehicle/15  "CM_Global_Ax"
  Demux/1023 -> Vehicle/16  "CM_Global_Ay"
  Demux/1024 -> Vehicle/17  "CM_Global_Vx"
  Demux/1025 -> Vehicle/18  "CM_Global_Vy"
  Demux/1026 -> Vehicle/19  "CM_Global_X"
  Demux/1027 -> Vehicle/20  "CM_Global_Y"
  Demux/1028 -> Vehicle/21  "CM_Global_Z"
  Demux/1029 -> Vehicle/22  "CM_Tracking_Ax"
  Demux/1030 -> Vehicle/23  "CM_Tracking_Ay"
  Demux/1031 -> Vehicle/24  "CM_Tracking_Vx"
  Demux/1032 -> Vehicle/25  "CM_Tracking_Vy"
  Demux/1033 -> Vehicle/26  "cross_weight_PID"
  Demux/1034 -> Vehicle/27  "Euler_Roll"
  Demux/1035 -> Vehicle/28  "front_ride_height_at_center_point"
  Demux/1036 -> Vehicle/29  "Global_Alpha_X"
  Demux/1037 -> Vehicle/30  "Global_Alpha_Y"
  Demux/1038 -> Vehicle/31  "Global_Alpha_Z"
  Demux/1039 -> Vehicle/32  "Global_Omega_X"
  Demux/1040 -> Vehicle/33  "Global_Omega_Y"
  Demux/1041 -> Vehicle/34  "Global_Omega_Z"
  Demux/1042 -> Vehicle/35  "Inclination_Roll"
  Demux/1043 -> Vehicle/36  "Origin_Distance_Traveled"
  Demux/1044 -> Vehicle/37  "Origin_Global_X"
  Demux/1045 -> Vehicle/38  "Origin_Global_Y"
  Demux/1046 -> Vehicle/39  "Origin_Global_Z"
  Demux/1047 -> Vehicle/40  "Origin_Global_Z_wrt_road_mk"
  Demux/1048 -> Vehicle/41  "Pitch"
  Demux/1049 -> Vehicle/42  "Side_Slip_Angle"
  Demux/1050 -> Vehicle/43  "Side_Slip_Angle_Rate"
  Demux/1051 -> Vehicle/44  "Understeer_Gradient"
  Demux/1052 -> Vehicle/45  "Understeer_Stability_Factor"
  Demux/1053 -> Vehicle/46  "Yaw"
  Vehicle_States/1 -> OutputBus/83  "Vehicle_States"
  Demux/1054 -> Vehicle_States/1  "horizontal_vel_wrt_road"
  Demux/1055 -> Vehicle_States/2  "lateral_acc_wrt_road"
  Demux/1056 -> Vehicle_States/3  "lateral_disp"
  Demux/1057 -> Vehicle_States/4  "lateral_vel_wrt_road"
  Demux/1058 -> Vehicle_States/5  "longitudinal_acc_wrt_road"
  Demux/1059 -> Vehicle_States/6  "longitudinal_disp"
  Demux/1060 -> Vehicle_States/7  "longitudinal_vel_wrt_road"
  Demux/1061 -> Vehicle_States/8  "pitch_angle"
  Demux/1062 -> Vehicle_States/9  "pitch_angular_acc_wrt_road"
  Demux/1063 -> Vehicle_States/10  "pitch_angular_vel_wrt_road"
  Demux/1064 -> Vehicle_States/11  "roll_angle"
  Demux/1065 -> Vehicle_States/12  "roll_angular_acc_wrt_road"
  Demux/1066 -> Vehicle_States/13  "roll_angular_vel_wrt_road"
  Demux/1067 -> Vehicle_States/14  "side_slip"
  Demux/1068 -> Vehicle_States/15  "vertical_acc_wrt_road"
  Demux/1069 -> Vehicle_States/16  "vertical_disp"
  Demux/1070 -> Vehicle_States/17  "vertical_vel_wrt_road"
  Demux/1071 -> Vehicle_States/18  "yaw_angle"
  Demux/1072 -> Vehicle_States/19  "yaw_angular_acc_wrt_road"
  Demux/1073 -> Vehicle_States/20  "yaw_angular_vel_wrt_road"
  Wheel/1 -> OutputBus/84  "Wheel"
  Alpha/1 -> Wheel/1  "Alpha"
  Demux/1074 -> Alpha/1  "L1"
  Demux/1075 -> Alpha/2  "L2"
  Demux/1076 -> Alpha/3  "R1"
  Demux/1077 -> Alpha/4  "R2"
  Caster_Angle/1 -> Wheel/2  "Caster_Angle"
  Demux/1078 -> Caster_Angle/1  "left"
  Demux/1079 -> Caster_Angle/2  "right"
  Drive_Moment/1 -> Wheel/3  "Drive_Moment"
  Demux/1080 -> Drive_Moment/1  "L1"
  Demux/1081 -> Drive_Moment/2  "L2"
  Demux/1082 -> Drive_Moment/3  "R1"
  Demux/1083 -> Drive_Moment/4  "R2"
  Euler_Roll/1 -> Wheel/4  "Euler_Roll"
  Demux/1084 -> Euler_Roll/1  "L1"
  Demux/1085 -> Euler_Roll/2  "L2"
  Demux/1086 -> Euler_Roll/3  "R1"
  Demux/1087 -> Euler_Roll/4  "R2"
  Global_Omega_X/1 -> Wheel/5  "Global_Omega_X"
  Demux/1088 -> Global_Omega_X/1  "L1"
  Demux/1089 -> Global_Omega_X/2  "L2"
  Demux/1090 -> Global_Omega_X/3  "R1"
  Demux/1091 -> Global_Omega_X/4  "R2"
  Global_Omega_Y/1 -> Wheel/6  "Global_Omega_Y"
  Demux/1092 -> Global_Omega_Y/1  "L1"
  Demux/1093 -> Global_Omega_Y/2  "L2"
  Demux/1094 -> Global_Omega_Y/3  "R1"
  Demux/1095 -> Global_Omega_Y/4  "R2"
  Global_Omega_Z/1 -> Wheel/7  "Global_Omega_Z"
  Demux/1096 -> Global_Omega_Z/1  "L1"
  Demux/1097 -> Global_Omega_Z/2  "L2"
  Demux/1098 -> Global_Omega_Z/3  "R1"
  Demux/1099 -> Global_Omega_Z/4  "R2"
  Global_Vx/1 -> Wheel/8  "Global_Vx"
  Demux/1100 -> Global_Vx/1  "L1"
  Demux/1101 -> Global_Vx/2  "L2"
  Demux/1102 -> Global_Vx/3  "R1"
  Demux/1103 -> Global_Vx/4  "R2"
  Global_Vy/1 -> Wheel/9  "Global_Vy"
  Demux/1104 -> Global_Vy/1  "L1"
  Demux/1105 -> Global_Vy/2  "L2"
  Demux/1106 -> Global_Vy/3  "R1"
  Demux/1107 -> Global_Vy/4  "R2"
  Global_Vz/1 -> Wheel/10  "Global_Vz"
  Demux/1108 -> Global_Vz/1  "L1"
  Demux/1109 -> Global_Vz/2  "L2"
  Demux/1110 -> Global_Vz/3  "R1"
  Demux/1111 -> Global_Vz/4  "R2"
  Global_X/1 -> Wheel/11  "Global_X"
  Demux/1112 -> Global_X/1  "L1"
  Demux/1113 -> Global_X/2  "L2"
  Demux/1114 -> Global_X/3  "R1"
  Demux/1115 -> Global_X/4  "R2"
  Global_Y/1 -> Wheel/12  "Global_Y"
  Demux/1116 -> Global_Y/1  "L1"
  Demux/1117 -> Global_Y/2  "L2"
  Demux/1118 -> Global_Y/3  "R1"
  Demux/1119 -> Global_Y/4  "R2"
  Global_Z/1 -> Wheel/13  "Global_Z"
  Demux/1120 -> Global_Z/1  "L1"
  Demux/1121 -> Global_Z/2  "L2"
  Demux/1122 -> Global_Z/3  "R1"
  Demux/1123 -> Global_Z/4  "R2"
  Ground_Surface_Wheel_Center_Vx/1 -> Wheel/14  "Ground_Surface_Wheel_Center_Vx"
  Demux/1124 -> Ground_Surface_Wheel_Center_Vx/1  "L1"
  Demux/1125 -> Ground_Surface_Wheel_Center_Vx/2  "L2"
  Demux/1126 -> Ground_Surface_Wheel_Center_Vx/3  "R1"
  Demux/1127 -> Ground_Surface_Wheel_Center_Vx/4  "R2"
  Hub_Carrier_Omega_X/1 -> Wheel/15  "Hub_Carrier_Omega_X"
  Demux/1128 -> Hub_Carrier_Omega_X/1  "L1"
  Demux/1129 -> Hub_Carrier_Omega_X/2  "L2"
  Demux/1130 -> Hub_Carrier_Omega_X/3  "R1"
  Demux/1131 -> Hub_Carrier_Omega_X/4  "R2"
  Hub_Carrier_Omega_Y/1 -> Wheel/16  "Hub_Carrier_Omega_Y"
  Demux/1132 -> Hub_Carrier_Omega_Y/1  "L1"
  Demux/1133 -> Hub_Carrier_Omega_Y/2  "L2"
  Demux/1134 -> Hub_Carrier_Omega_Y/3  "R1"
  Demux/1135 -> Hub_Carrier_Omega_Y/4  "R2"
  Hub_Carrier_Omega_Z/1 -> Wheel/17  "Hub_Carrier_Omega_Z"
  Demux/1136 -> Hub_Carrier_Omega_Z/1  "L1"
  Demux/1137 -> Hub_Carrier_Omega_Z/2  "L2"
  Demux/1138 -> Hub_Carrier_Omega_Z/3  "R1"
  Demux/1139 -> Hub_Carrier_Omega_Z/4  "R2"
  Hub_Carrier_Vx/1 -> Wheel/18  "Hub_Carrier_Vx"
  Demux/1140 -> Hub_Carrier_Vx/1  "L1"
  Demux/1141 -> Hub_Carrier_Vx/2  "L2"
  Demux/1142 -> Hub_Carrier_Vx/3  "R1"
  Demux/1143 -> Hub_Carrier_Vx/4  "R2"
  Hub_Carrier_Vy/1 -> Wheel/19  "Hub_Carrier_Vy"
  Demux/1144 -> Hub_Carrier_Vy/1  "L1"
  Demux/1145 -> Hub_Carrier_Vy/2  "L2"
  Demux/1146 -> Hub_Carrier_Vy/3  "R1"
  Demux/1147 -> Hub_Carrier_Vy/4  "R2"
  Hub_Carrier_Vz/1 -> Wheel/20  "Hub_Carrier_Vz"
  Demux/1148 -> Hub_Carrier_Vz/1  "L1"
  Demux/1149 -> Hub_Carrier_Vz/2  "L2"
  Demux/1150 -> Hub_Carrier_Vz/3  "R1"
  Demux/1151 -> Hub_Carrier_Vz/4  "R2"
  hub_center_accx/1 -> Wheel/21  "hub_center_accx"
  Demux/1152 -> hub_center_accx/1  "front_left"
  Demux/1153 -> hub_center_accx/2  "front_right"
  Demux/1154 -> hub_center_accx/3  "rear_left"
  Demux/1155 -> hub_center_accx/4  "rear_right"
  hub_center_accy/1 -> Wheel/22  "hub_center_accy"
  Demux/1156 -> hub_center_accy/1  "front_left"
  Demux/1157 -> hub_center_accy/2  "front_right"
  Demux/1158 -> hub_center_accy/3  "rear_left"
  Demux/1159 -> hub_center_accy/4  "rear_right"
  hub_center_accz/1 -> Wheel/23  "hub_center_accz"
  Demux/1160 -> hub_center_accz/1  "front_left"
  Demux/1161 -> hub_center_accz/2  "front_right"
  Demux/1162 -> hub_center_accz/3  "rear_left"
  Demux/1163 -> hub_center_accz/4  "rear_right"
  Inclination/1 -> Wheel/24  "Inclination"
  Demux/1164 -> Inclination/1  "L1"
  Demux/1165 -> Inclination/2  "L2"
  Demux/1166 -> Inclination/3  "R1"
  Demux/1167 -> Inclination/4  "R2"
  Kingpin_Moment1/1 -> Wheel/25  "Kingpin_Moment"
  Demux/1168 -> Kingpin_Moment1/1  "L1"
  Demux/1169 -> Kingpin_Moment1/2  "R1"
  Omega/1 -> Wheel/26  "Omega"
  Demux/1170 -> Omega/1  "L1"
  Demux/1171 -> Omega/2  "L2"
  Demux/1172 -> Omega/3  "R1"
  Demux/1173 -> Omega/4  "R2"
  Phi/1 -> Wheel/27  "Phi"
  Demux/1174 -> Phi/1  "L1"
  Demux/1175 -> Phi/2  "L2"
  Demux/1176 -> Phi/3  "R1"
  Demux/1177 -> Phi/4  "R2"
  Pitch/1 -> Wheel/28  "Pitch"
  Demux/1178 -> Pitch/1  "L1"
  Demux/1179 -> Pitch/2  "L2"
  Demux/1180 -> Pitch/3  "R1"
  Demux/1181 -> Pitch/4  "R2"
  Psi/1 -> Wheel/29  "Psi"
  Demux/1182 -> Psi/1  "L1"
  Demux/1183 -> Psi/2  "L2"
  Demux/1184 -> Psi/3  "R1"
  Demux/1185 -> Psi/4  "R2"
  Rotation/1 -> Wheel/30  "Rotation"
  Demux/1186 -> Rotation/1  "L1"
  Demux/1187 -> Rotation/2  "L2"
  Demux/1188 -> Rotation/3  "R1"
  Demux/1189 -> Rotation/4  "R2"
  Side_View_Angle/1 -> Wheel/31  "Side_View_Angle"
  Demux/1190 -> Side_View_Angle/1  "L1"
  Demux/1191 -> Side_View_Angle/2  "L2"
  Demux/1192 -> Side_View_Angle/3  "R1"
  Demux/1193 -> Side_View_Angle/4  "R2"
  Spindle_Steer/1 -> Wheel/32  "Spindle_Steer"
  Demux/1194 -> Spindle_Steer/1  "L1"
  Demux/1195 -> Spindle_Steer/2  "L2"
  Demux/1196 -> Spindle_Steer/3  "R1"
  Demux/1197 -> Spindle_Steer/4  "R2"
  Theta/1 -> Wheel/33  "Theta"
  Demux/1198 -> Theta/1  "L1"
  Demux/1199 -> Theta/2  "L2"
  Demux/1200 -> Theta/3  "R1"
  Demux/1201 -> Theta/4  "R2"
  wheel_center_dispx/1 -> Wheel/34  "wheel_center_dispx"
  Demux/1202 -> wheel_center_dispx/1  "front_left"
  Demux/1203 -> wheel_center_dispx/2  "front_right"
  Demux/1204 -> wheel_center_dispx/3  "rear_left"
  Demux/1205 -> wheel_center_dispx/4  "rear_right"
  wheel_center_dispy/1 -> Wheel/35  "wheel_center_dispy"
  Demux/1206 -> wheel_center_dispy/1  "front_left"
  Demux/1207 -> wheel_center_dispy/2  "front_right"
  Demux/1208 -> wheel_center_dispy/3  "rear_left"
  Demux/1209 -> wheel_center_dispy/4  "rear_right"
  wheel_center_dispz/1 -> Wheel/36  "wheel_center_dispz"
  Demux/1210 -> wheel_center_dispz/1  "front_left"
  Demux/1211 -> wheel_center_dispz/2  "front_right"
  Demux/1212 -> wheel_center_dispz/3  "rear_left"
  Demux/1213 -> wheel_center_dispz/4  "rear_right"
  Yaw/1 -> Wheel/37  "Yaw"
  Demux/1214 -> Yaw/1  "L1"
  Demux/1215 -> Yaw/2  "L2"
  Demux/1216 -> Yaw/3  "R1"
  Demux/1217 -> Yaw/4  "R2"
  wheel_angles/1 -> OutputBus/85  "wheel_angles"
  Demux/1218 -> wheel_angles/1  "camber_L1"
  Demux/1219 -> wheel_angles/2  "camber_L2"
  Demux/1220 -> wheel_angles/3  "camber_R1"
  Demux/1221 -> wheel_angles/4  "camber_R2"
  Demux/1222 -> wheel_angles/5  "camber_wrt_road_L1"
  Demux/1223 -> wheel_angles/6  "camber_wrt_road_L2"
  Demux/1224 -> wheel_angles/7  "camber_wrt_road_R1"
  Demux/1225 -> wheel_angles/8  "camber_wrt_road_R2"
  Demux/1226 -> wheel_angles/9  "caster_L1"
  Demux/1227 -> wheel_angles/10  "caster_L2"
  Demux/1228 -> wheel_angles/11  "caster_R1"
  Demux/1229 -> wheel_angles/12  "caster_R2"
  Demux/1230 -> wheel_angles/13  "caster_wrt_road_L1"
  Demux/1231 -> wheel_angles/14  "caster_wrt_road_L2"
  Demux/1232 -> wheel_angles/15  "caster_wrt_road_R1"
  Demux/1233 -> wheel_angles/16  "caster_wrt_road_R2"
  Demux/1234 -> wheel_angles/17  "toe_L1"
  Demux/1235 -> wheel_angles/18  "toe_L2"
  Demux/1236 -> wheel_angles/19  "toe_R1"
  Demux/1237 -> wheel_angles/20  "toe_R2"
  Demux/1238 -> wheel_angles/21  "toe_wrt_road_L1"
  Demux/1239 -> wheel_angles/22  "toe_wrt_road_L2"
  Demux/1240 -> wheel_angles/23  "toe_wrt_road_R1"
  Demux/1241 -> wheel_angles/24  "toe_wrt_road_R2"
  whl_front_wheel_XFORM/1 -> OutputBus/86  "whl_front_wheel_XFORM"
  Demux/1242 -> whl_front_wheel_XFORM/1  "FX"
  Demux/1243 -> whl_front_wheel_XFORM/2  "FY"
  Demux/1244 -> whl_front_wheel_XFORM/3  "FZ"
  Demux/1245 -> whl_front_wheel_XFORM/4  "Phi"
  Demux/1246 -> whl_front_wheel_XFORM/5  "Psi"
  Demux/1247 -> whl_front_wheel_XFORM/6  "Theta"
  Demux/1248 -> whl_front_wheel_XFORM/7  "X"
  Demux/1249 -> whl_front_wheel_XFORM/8  "Y"
  Demux/1250 -> whl_front_wheel_XFORM/9  "Z"
  whl_rear_wheel_XFORM/1 -> OutputBus/87  "whl_rear_wheel_XFORM"
  Demux/1251 -> whl_rear_wheel_XFORM/1  "FX"
  Demux/1252 -> whl_rear_wheel_XFORM/2  "FY"
  Demux/1253 -> whl_rear_wheel_XFORM/3  "FZ"
  Demux/1254 -> whl_rear_wheel_XFORM/4  "Phi"
  Demux/1255 -> whl_rear_wheel_XFORM/5  "Psi"
  Demux/1256 -> whl_rear_wheel_XFORM/6  "Theta"
  Demux/1257 -> whl_rear_wheel_XFORM/7  "X"
  Demux/1258 -> whl_rear_wheel_XFORM/8  "Y"
  Demux/1259 -> whl_rear_wheel_XFORM/9  "Z"
  whl_twin_rear_wheel_XFORM/1 -> OutputBus/88  "whl_twin_rear_wheel_XFORM"
  Demux/1260 -> whl_twin_rear_wheel_XFORM/1  "FX"
  Demux/1261 -> whl_twin_rear_wheel_XFORM/2  "FY"
  Demux/1262 -> whl_twin_rear_wheel_XFORM/3  "FZ"
  Demux/1263 -> whl_twin_rear_wheel_XFORM/4  "Phi"
  Demux/1264 -> whl_twin_rear_wheel_XFORM/5  "Psi"
  Demux/1265 -> whl_twin_rear_wheel_XFORM/6  "Theta"
  Demux/1266 -> whl_twin_rear_wheel_XFORM/7  "X"
  Demux/1267 -> whl_twin_rear_wheel_XFORM/8  "Y"
  Demux/1268 -> whl_twin_rear_wheel_XFORM/9  "Z"
  whr_front_wheel_XFORM/1 -> OutputBus/89  "whr_front_wheel_XFORM"
  Demux/1269 -> whr_front_wheel_XFORM/1  "FX"
  Demux/1270 -> whr_front_wheel_XFORM/2  "FY"
  Demux/1271 -> whr_front_wheel_XFORM/3  "FZ"
  Demux/1272 -> whr_front_wheel_XFORM/4  "Phi"
  Demux/1273 -> whr_front_wheel_XFORM/5  "Psi"
  Demux/1274 -> whr_front_wheel_XFORM/6  "Theta"
  Demux/1275 -> whr_front_wheel_XFORM/7  "X"
  Demux/1276 -> whr_front_wheel_XFORM/8  "Y"
  Demux/1277 -> whr_front_wheel_XFORM/9  "Z"
  whr_rear_wheel_XFORM/1 -> OutputBus/90  "whr_rear_wheel_XFORM"
  Demux/1278 -> whr_rear_wheel_XFORM/1  "FX"
  Demux/1279 -> whr_rear_wheel_XFORM/2  "FY"
  Demux/1280 -> whr_rear_wheel_XFORM/3  "FZ"
  Demux/1281 -> whr_rear_wheel_XFORM/4  "Phi"
  Demux/1282 -> whr_rear_wheel_XFORM/5  "Psi"
  Demux/1283 -> whr_rear_wheel_XFORM/6  "Theta"
  Demux/1284 -> whr_rear_wheel_XFORM/7  "X"
  Demux/1285 -> whr_rear_wheel_XFORM/8  "Y"
  Demux/1286 -> whr_rear_wheel_XFORM/9  "Z"
  whr_twin_rear_wheel_XFORM/1 -> OutputBus/91  "whr_twin_rear_wheel_XFORM"
  Demux/1287 -> whr_twin_rear_wheel_XFORM/1  "FX"
  Demux/1288 -> whr_twin_rear_wheel_XFORM/2  "FY"
  Demux/1289 -> whr_twin_rear_wheel_XFORM/3  "FZ"
  Demux/1290 -> whr_twin_rear_wheel_XFORM/4  "Phi"
  Demux/1291 -> whr_twin_rear_wheel_XFORM/5  "Psi"
  Demux/1292 -> whr_twin_rear_wheel_XFORM/6  "Theta"
  Demux/1293 -> whr_twin_rear_wheel_XFORM/7  "X"
  Demux/1294 -> whr_twin_rear_wheel_XFORM/8  "Y"
  Demux/1295 -> whr_twin_rear_wheel_XFORM/9  "Z"
  Animator_Widget/1 -> OutputBus/92  "Animator_Widget"
  Demux/1296 -> Animator_Widget/1  "longitudinal_speed"
  Demux/1297 -> Animator_Widget/2  "engine_rpm"
  ges_hub_XFORMFL/1 -> OutputBus/93  "ges_hub_XFORMFL"
  Demux/1299 -> ges_hub_XFORMFL/1  "X"
  Demux/1300 -> ges_hub_XFORMFL/2  "Y"
  Demux/1301 -> ges_hub_XFORMFL/3  "Z"
  Demux/1302 -> ges_hub_XFORMFL/4  "Psi"
  Demux/1303 -> ges_hub_XFORMFL/5  "Theta"
  Demux/1304 -> ges_hub_XFORMFL/6  "Phi"
  hub2cp_XFORMFL/1 -> OutputBus/94  "hub2cp_XFORMFL"
  Demux/1305 -> hub2cp_XFORMFL/1  "X"
  Demux/1306 -> hub2cp_XFORMFL/2  "Y"
  Demux/1307 -> hub2cp_XFORMFL/3  "Z"
  cp_force_longitudinalFL/1 -> OutputBus/95  "cp_force_longitudinalFL"
  Demux/1308 -> cp_force_longitudinalFL/1  "X"
  Demux/1309 -> cp_force_longitudinalFL/2  "Y"
  Demux/1310 -> cp_force_longitudinalFL/3  "Z"
  cp_force_lateralFL/1 -> OutputBus/96  "cp_force_lateralFL"
  Demux/1311 -> cp_force_lateralFL/1  "X"
  Demux/1312 -> cp_force_lateralFL/2  "Y"
  Demux/1313 -> cp_force_lateralFL/3  "Z"
  cp_force_normalFL/1 -> OutputBus/97  "cp_force_normalFL"
  Demux/1314 -> cp_force_normalFL/1  "X"
  Demux/1315 -> cp_force_normalFL/2  "Y"
  Demux/1316 -> cp_force_normalFL/3  "Z"
  ges_hub_XFORMFR/1 -> OutputBus/98  "ges_hub_XFORMFR"
  Demux/1317 -> ges_hub_XFORMFR/1  "X"
  Demux/1318 -> ges_hub_XFORMFR/2  "Y"
  Demux/1319 -> ges_hub_XFORMFR/3  "Z"
  Demux/1320 -> ges_hub_XFORMFR/4  "Psi"
  Demux/1321 -> ges_hub_XFORMFR/5  "Theta"
  Demux/1322 -> ges_hub_XFORMFR/6  "Phi"
  hub2cp_XFORMFR/1 -> OutputBus/99  "hub2cp_XFORMFR"
  Demux/1323 -> hub2cp_XFORMFR/1  "X"
  Demux/1324 -> hub2cp_XFORMFR/2  "Y"
  Demux/1325 -> hub2cp_XFORMFR/3  "Z"
  cp_force_longitudinalFR/1 -> OutputBus/100  "cp_force_longitudinalFR"
  Demux/1326 -> cp_force_longitudinalFR/1  "X"
  Demux/1327 -> cp_force_longitudinalFR/2  "Y"
  Demux/1328 -> cp_force_longitudinalFR/3  "Z"
  cp_force_lateralFR/1 -> OutputBus/101  "cp_force_lateralFR"
  Demux/1329 -> cp_force_lateralFR/1  "X"
  Demux/1330 -> cp_force_lateralFR/2  "Y"
  Demux/1331 -> cp_force_lateralFR/3  "Z"
  cp_force_normalFR/1 -> OutputBus/102  "cp_force_normalFR"
  Demux/1332 -> cp_force_normalFR/1  "X"
  Demux/1333 -> cp_force_normalFR/2  "Y"
  Demux/1334 -> cp_force_normalFR/3  "Z"
  ges_hub_XFORMRL/1 -> OutputBus/103  "ges_hub_XFORMRL"
  Demux/1335 -> ges_hub_XFORMRL/1  "X"
  Demux/1336 -> ges_hub_XFORMRL/2  "Y"
  Demux/1337 -> ges_hub_XFORMRL/3  "Z"
  Demux/1338 -> ges_hub_XFORMRL/4  "Psi"
  Demux/1339 -> ges_hub_XFORMRL/5  "Theta"
  Demux/1340 -> ges_hub_XFORMRL/6  "Phi"
  hub2cp_XFORMRL/1 -> OutputBus/104  "hub2cp_XFORMRL"
  Demux/1341 -> hub2cp_XFORMRL/1  "X"
  Demux/1342 -> hub2cp_XFORMRL/2  "Y"
  Demux/1343 -> hub2cp_XFORMRL/3  "Z"
  cp_force_longitudinalRL/1 -> OutputBus/105  "cp_force_longitudinalRL"
  Demux/1344 -> cp_force_longitudinalRL/1  "X"
  Demux/1345 -> cp_force_longitudinalRL/2  "Y"
  Demux/1346 -> cp_force_longitudinalRL/3  "Z"
  cp_force_lateralRL/1 -> OutputBus/106  "cp_force_lateralRL"
  Demux/1347 -> cp_force_lateralRL/1  "X"
  Demux/1348 -> cp_force_lateralRL/2  "Y"
  Demux/1349 -> cp_force_lateralRL/3  "Z"
  cp_force_normalRL/1 -> OutputBus/107  "cp_force_normalRL"
  Demux/1350 -> cp_force_normalRL/1  "X"
  Demux/1351 -> cp_force_normalRL/2  "Y"
  Demux/1352 -> cp_force_normalRL/3  "Z"
  ges_hub_XFORMRR/1 -> OutputBus/108  "ges_hub_XFORMRR"
  Demux/1353 -> ges_hub_XFORMRR/1  "X"
  Demux/1354 -> ges_hub_XFORMRR/2  "Y"
  Demux/1355 -> ges_hub_XFORMRR/3  "Z"
  Demux/1356 -> ges_hub_XFORMRR/4  "Psi"
  Demux/1357 -> ges_hub_XFORMRR/5  "Theta"
  Demux/1358 -> ges_hub_XFORMRR/6  "Phi"
  hub2cp_XFORMRR/1 -> OutputBus/109  "hub2cp_XFORMRR"
  Demux/1359 -> hub2cp_XFORMRR/1  "X"
  Demux/1360 -> hub2cp_XFORMRR/2  "Y"
  Demux/1361 -> hub2cp_XFORMRR/3  "Z"
  cp_force_longitudinalRR/1 -> OutputBus/110  "cp_force_longitudinalRR"
  Demux/1362 -> cp_force_longitudinalRR/1  "X"
  Demux/1363 -> cp_force_longitudinalRR/2  "Y"
  Demux/1364 -> cp_force_longitudinalRR/3  "Z"
  cp_force_lateralRR/1 -> OutputBus/111  "cp_force_lateralRR"
  Demux/1365 -> cp_force_lateralRR/1  "X"
  Demux/1366 -> cp_force_lateralRR/2  "Y"
  Demux/1367 -> cp_force_lateralRR/3  "Z"
  cp_force_normalRR/1 -> OutputBus/112  "cp_force_normalRR"
  Demux/1368 -> cp_force_normalRR/1  "X"
  Demux/1369 -> cp_force_normalRR/2  "Y"
  Demux/1370 -> cp_force_normalRR/3  "Z"
  Road_Material/1 -> OutputBus/113  "Road_Material"
  Demux/1371 -> Road_Material/1  "front_left_tire"
  Demux/1372 -> Road_Material/2  "front_right_tire"
  Demux/1373 -> Road_Material/3  "rear_left_tire"
  Demux/1374 -> Road_Material/4  "rear_right_tire"
